simulink model "OR_10s_70l"  (R2023b)
settings: Solver=VariableStepAuto  StartTime=0.0  StopTime=10.0  RelTol=1e-3
undefined symbols (not defined in the file or in its folder): null
libraries: ABB_UPPAAL_Library x168
(part 1 of 3)
settings Model: Creator=francescopellei  LastModifiedBy=francescopellei

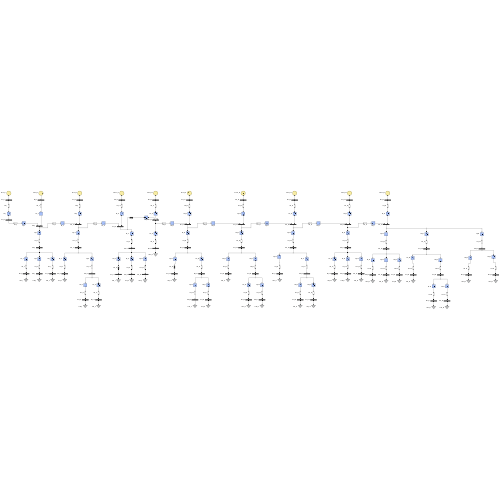
[thumbnail: Simulink's stored preview of the top-level diagram]
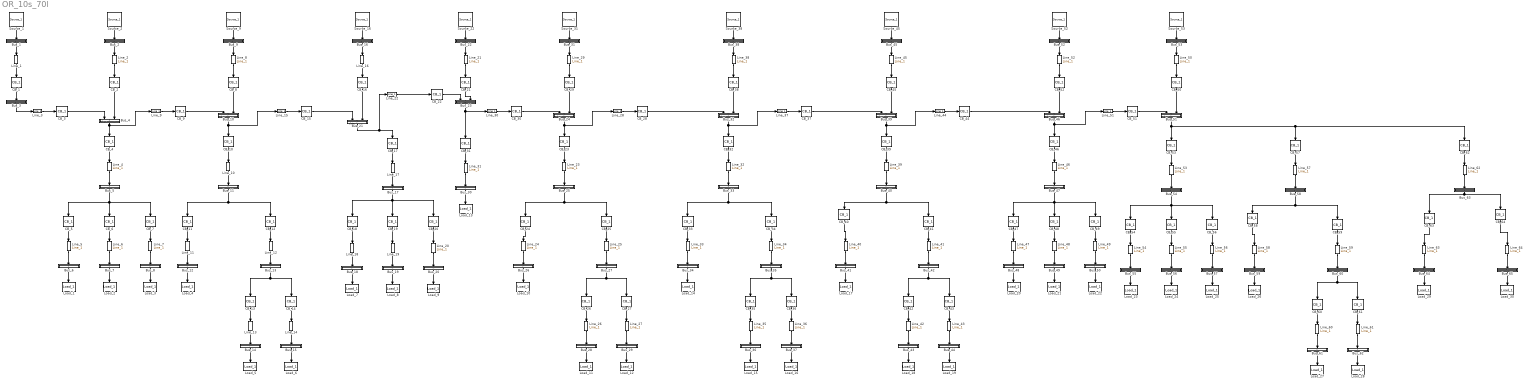
== system OR_10s_70l ==
  Bus_1 : MATLAB Function  TreatAsAtomicUnit=on  mask{MyInitialization=0, Bus_ID=1, Fault_flag=1}
      mask prompts: Bus_ID "Bus ID"; Fault_flag "Fault flag"
      settings: CopyFcn=|
      | Component_Name = get_param(gcb, 'Name');
      | set_param(gcb, 'Bus_ID', num2str(strtrim(extractAfter(Component_Name, '_'))));
      | 
      | blocks = find_system(gcs, 'SearchDepth', 1, 'Type', 'Block');
      | 
      | for k = 1:length(blocks)
      |     if contains(extractAfter(blocks{k,1}, '/'), 'Source')
      |         set_param(blocks{k}, 'BackgroundColor', '[0.929000, 0.490000, 0.439000]');
      |     end
      | end
      settings: NameChangeFcn=|
      | Component_Name = get_param(gcb, 'Name');
      | old_ID = get_param(gcb, 'Bus_ID');
      | 
      | pattern = '_\d+';
      | match = regexp(Component_Name, pattern, 'match');
      | 
      | if ~isempty(match)
      |     if ~isequal(old_ID, num2str(strtrim(extractAfter(Component_Name, '_'))))
      |         set_param(gcb, 'Bus_ID', num2str(strtrim(extractAfter(Component_Name, '_'))));
      |     end
      | else
      |     newName = [Component_Name '_' old_ID];
      |     set_param(gcb, 'Name', newName);
      | end
      | 
      | if ~isequal(old_ID, get_param(gcb, 'Bus_ID'))
      | 
      |     data = get_param(gcb, 'PortConnectivity');
      |     for i = 1:numel(data)
      |         sourceHandle = data(i,1).SrcBlock;
      |         if ~isempty(sourceHandle) && sourceHandle ~= -1
      |             sourceParams = get_param(sourceHandle, 'DialogParameters');
      |             fn = fieldnames(sourceParams);
      |             if contains(fn{2}, 'Source')
      |                 Bus_ID = get_param(gcb, 'Bus_ID');
      |                 set_param(sourceHandle, 'Source_ID', Bus_ID);
      |             end
      |         end
      |     end
      | 
      |     blocks = find_system(gcs, 'SearchDepth', 1, 'Type', 'Block');
      | 
      |     for k = 1:length(blocks)
      |         if contains(extractAfter(blocks{k,1}, '/'), 'Source')
      |             set_param(blocks{k}, 'BackgroundColor', '[0.929000, 0.490000, 0.439000]');
      |         end
      |     end
      | 
      | end
      settings: PreDeleteFcn=|
      | blocks = find_system(gcs, 'SearchDepth', 1, 'Type', 'Block');
      | 
      | for k = 1:length(blocks)
      |     if contains(extractAfter(blocks{k,1}, '/'), 'Source')
      |         set_param(blocks{k}, 'BackgroundColor', '[0.929000, 0.490000, 0.439000]');
      |     end
      | end
  Bus_10 : MATLAB Function  TreatAsAtomicUnit=on  mask{MyInitialization=0, Bus_ID=10, Fault_flag=1}
      mask prompts: Bus_ID "Bus ID"; Fault_flag "Fault flag"
      settings: CopyFcn=|
      | Component_Name = get_param(gcb, 'Name');
      | set_param(gcb, 'Bus_ID', num2str(strtrim(extractAfter(Component_Name, '_'))));
      | 
      | blocks = find_system(gcs, 'SearchDepth', 1, 'Type', 'Block');
      | 
      | for k = 1:length(blocks)
      |     if contains(extractAfter(blocks{k,1}, '/'), 'Source')
      |         set_param(blocks{k}, 'BackgroundColor', '[0.929000, 0.490000, 0.439000]');
      |     end
      | end
      settings: NameChangeFcn=|
      | Component_Name = get_param(gcb, 'Name');
      | old_ID = get_param(gcb, 'Bus_ID');
      | 
      | pattern = '_\d+';
      | match = regexp(Component_Name, pattern, 'match');
      | 
      | if ~isempty(match)
      |     if ~isequal(old_ID, num2str(strtrim(extractAfter(Component_Name, '_'))))
      |         set_param(gcb, 'Bus_ID', num2str(strtrim(extractAfter(Component_Name, '_'))));
      |     end
      | else
      |     newName = [Component_Name '_' old_ID];
      |     set_param(gcb, 'Name', newName);
      | end
      | 
      | if ~isequal(old_ID, get_param(gcb, 'Bus_ID'))
      | 
      |     data = get_param(gcb, 'PortConnectivity');
      |     for i = 1:numel(data)
      |         sourceHandle = data(i,1).SrcBlock;
      |         if ~isempty(sourceHandle) && sourceHandle ~= -1
      |             sourceParams = get_param(sourceHandle, 'DialogParameters');
      |             fn = fieldnames(sourceParams);
      |             if contains(fn{2}, 'Source')
      |                 Bus_ID = get_param(gcb, 'Bus_ID');
      |                 set_param(sourceHandle, 'Source_ID', Bus_ID);
      |             end
      |         end
      |     end
      | 
      |     blocks = find_system(gcs, 'SearchDepth', 1, 'Type', 'Block');
      | 
      |     for k = 1:length(blocks)
      |         if contains(extractAfter(blocks{k,1}, '/'), 'Source')
      |             set_param(blocks{k}, 'BackgroundColor', '[0.929000, 0.490000, 0.439000]');
      |         end
      |     end
      | 
      | end
      settings: PreDeleteFcn=|
      | blocks = find_system(gcs, 'SearchDepth', 1, 'Type', 'Block');
      | 
      | for k = 1:length(blocks)
      |     if contains(extractAfter(blocks{k,1}, '/'), 'Source')
      |         set_param(blocks{k}, 'BackgroundColor', '[0.929000, 0.490000, 0.439000]');
      |     end
      | end
  Bus_11 : MATLAB Function  TreatAsAtomicUnit=on  mask{MyInitialization=0, Bus_ID=11, Fault_flag=0}
      mask prompts: Bus_ID "Bus ID"; Fault_flag "Fault flag"
      settings: CopyFcn=|
      | Component_Name = get_param(gcb, 'Name');
      | set_param(gcb, 'Bus_ID', num2str(strtrim(extractAfter(Component_Name, '_'))));
      | 
      | blocks = find_system(gcs, 'SearchDepth', 1, 'Type', 'Block');
      | 
      | for k = 1:length(blocks)
      |     if contains(extractAfter(blocks{k,1}, '/'), 'Source')
      |         set_param(blocks{k}, 'BackgroundColor', '[0.929000, 0.490000, 0.439000]');
      |     end
      | end
      settings: NameChangeFcn=|
      | Component_Name = get_param(gcb, 'Name');
      | old_ID = get_param(gcb, 'Bus_ID');
      | 
      | pattern = '_\d+';
      | match = regexp(Component_Name, pattern, 'match');
      | 
      | if ~isempty(match)
      |     if ~isequal(old_ID, num2str(strtrim(extractAfter(Component_Name, '_'))))
      |         set_param(gcb, 'Bus_ID', num2str(strtrim(extractAfter(Component_Name, '_'))));
      |     end
      | else
      |     newName = [Component_Name '_' old_ID];
      |     set_param(gcb, 'Name', newName);
      | end
      | 
      | if ~isequal(old_ID, get_param(gcb, 'Bus_ID'))
      | 
      |     data = get_param(gcb, 'PortConnectivity');
      |     for i = 1:numel(data)
      |         sourceHandle = data(i,1).SrcBlock;
      |         if ~isempty(sourceHandle) && sourceHandle ~= -1
      |             sourceParams = get_param(sourceHandle, 'DialogParameters');
      |             fn = fieldnames(sourceParams);
      |             if contains(fn{2}, 'Source')
      |                 Bus_ID = get_param(gcb, 'Bus_ID');
      |                 set_param(sourceHandle, 'Source_ID', Bus_ID);
      |             end
      |         end
      |     end
      | 
      |     blocks = find_system(gcs, 'SearchDepth', 1, 'Type', 'Block');
      | 
      |     for k = 1:length(blocks)
      |         if contains(extractAfter(blocks{k,1}, '/'), 'Source')
      |             set_param(blocks{k}, 'BackgroundColor', '[0.929000, 0.490000, 0.439000]');
      |         end
      |     end
      | 
      | end
      settings: PreDeleteFcn=|
      | blocks = find_system(gcs, 'SearchDepth', 1, 'Type', 'Block');
      | 
      | for k = 1:length(blocks)
      |     if contains(extractAfter(blocks{k,1}, '/'), 'Source')
      |         set_param(blocks{k}, 'BackgroundColor', '[0.929000, 0.490000, 0.439000]');
      |     end
      | end
  Bus_12 : MATLAB Function  TreatAsAtomicUnit=on  mask{MyInitialization=0, Bus_ID=12, Fault_flag=1}
      mask prompts: Bus_ID "Bus ID"; Fault_flag "Fault flag"
      settings: CopyFcn=|
      | Component_Name = get_param(gcb, 'Name');
      | set_param(gcb, 'Bus_ID', num2str(strtrim(extractAfter(Component_Name, '_'))));
      | 
      | blocks = find_system(gcs, 'SearchDepth', 1, 'Type', 'Block');
      | 
      | for k = 1:length(blocks)
      |     if contains(extractAfter(blocks{k,1}, '/'), 'Source')
      |         set_param(blocks{k}, 'BackgroundColor', '[0.929000, 0.490000, 0.439000]');
      |     end
      | end
      settings: NameChangeFcn=|
      | Component_Name = get_param(gcb, 'Name');
      | old_ID = get_param(gcb, 'Bus_ID');
      | 
      | pattern = '_\d+';
      | match = regexp(Component_Name, pattern, 'match');
      | 
      | if ~isempty(match)
      |     if ~isequal(old_ID, num2str(strtrim(extractAfter(Component_Name, '_'))))
      |         set_param(gcb, 'Bus_ID', num2str(strtrim(extractAfter(Component_Name, '_'))));
      |     end
      | else
      |     newName = [Component_Name '_' old_ID];
      |     set_param(gcb, 'Name', newName);
      | end
      | 
      | if ~isequal(old_ID, get_param(gcb, 'Bus_ID'))
      | 
      |     data = get_param(gcb, 'PortConnectivity');
      |     for i = 1:numel(data)
      |         sourceHandle = data(i,1).SrcBlock;
      |         if ~isempty(sourceHandle) && sourceHandle ~= -1
      |             sourceParams = get_param(sourceHandle, 'DialogParameters');
      |             fn = fieldnames(sourceParams);
      |             if contains(fn{2}, 'Source')
      |                 Bus_ID = get_param(gcb, 'Bus_ID');
      |                 set_param(sourceHandle, 'Source_ID', Bus_ID);
      |             end
      |         end
      |     end
      | 
      |     blocks = find_system(gcs, 'SearchDepth', 1, 'Type', 'Block');
      | 
      |     for k = 1:length(blocks)
      |         if contains(extractAfter(blocks{k,1}, '/'), 'Source')
      |             set_param(blocks{k}, 'BackgroundColor', '[0.929000, 0.490000, 0.439000]');
      |         end
      |     end
      | 
      | end
      settings: PreDeleteFcn=|
      | blocks = find_system(gcs, 'SearchDepth', 1, 'Type', 'Block');
      | 
      | for k = 1:length(blocks)
      |     if contains(extractAfter(blocks{k,1}, '/'), 'Source')
      |         set_param(blocks{k}, 'BackgroundColor', '[0.929000, 0.490000, 0.439000]');
      |     end
      | end
  Bus_13 : MATLAB Function  TreatAsAtomicUnit=on  mask{MyInitialization=0, Bus_ID=13, Fault_flag=1}
      mask prompts: Bus_ID "Bus ID"; Fault_flag "Fault flag"
      settings: CopyFcn=|
      | Component_Name = get_param(gcb, 'Name');
      | set_param(gcb, 'Bus_ID', num2str(strtrim(extractAfter(Component_Name, '_'))));
      | 
      | blocks = find_system(gcs, 'SearchDepth', 1, 'Type', 'Block');
      | 
      | for k = 1:length(blocks)
      |     if contains(extractAfter(blocks{k,1}, '/'), 'Source')
      |         set_param(blocks{k}, 'BackgroundColor', '[0.929000, 0.490000, 0.439000]');
      |     end
      | end
      settings: NameChangeFcn=|
      | Component_Name = get_param(gcb, 'Name');
      | old_ID = get_param(gcb, 'Bus_ID');
      | 
      | pattern = '_\d+';
      | match = regexp(Component_Name, pattern, 'match');
      | 
      | if ~isempty(match)
      |     if ~isequal(old_ID, num2str(strtrim(extractAfter(Component_Name, '_'))))
      |         set_param(gcb, 'Bus_ID', num2str(strtrim(extractAfter(Component_Name, '_'))));
      |     end
      | else
      |     newName = [Component_Name '_' old_ID];
      |     set_param(gcb, 'Name', newName);
      | end
      | 
      | if ~isequal(old_ID, get_param(gcb, 'Bus_ID'))
      | 
      |     data = get_param(gcb, 'PortConnectivity');
      |     for i = 1:numel(data)
      |         sourceHandle = data(i,1).SrcBlock;
      |         if ~isempty(sourceHandle) && sourceHandle ~= -1
      |             sourceParams = get_param(sourceHandle, 'DialogParameters');
      |             fn = fieldnames(sourceParams);
      |             if contains(fn{2}, 'Source')
      |                 Bus_ID = get_param(gcb, 'Bus_ID');
      |                 set_param(sourceHandle, 'Source_ID', Bus_ID);
      |             end
      |         end
      |     end
      | 
      |     blocks = find_system(gcs, 'SearchDepth', 1, 'Type', 'Block');
      | 
      |     for k = 1:length(blocks)
      |         if contains(extractAfter(blocks{k,1}, '/'), 'Source')
      |             set_param(blocks{k}, 'BackgroundColor', '[0.929000, 0.490000, 0.439000]');
      |         end
      |     end
      | 
      | end
      settings: PreDeleteFcn=|
      | blocks = find_system(gcs, 'SearchDepth', 1, 'Type', 'Block');
      | 
      | for k = 1:length(blocks)
      |     if contains(extractAfter(blocks{k,1}, '/'), 'Source')
      |         set_param(blocks{k}, 'BackgroundColor', '[0.929000, 0.490000, 0.439000]');
      |     end
      | end
  Bus_14 : MATLAB Function  TreatAsAtomicUnit=on  mask{MyInitialization=0, Bus_ID=14, Fault_flag=1}
      mask prompts: Bus_ID "Bus ID"; Fault_flag "Fault flag"
      settings: CopyFcn=|
      | Component_Name = get_param(gcb, 'Name');
      | set_param(gcb, 'Bus_ID', num2str(strtrim(extractAfter(Component_Name, '_'))));
      | 
      | blocks = find_system(gcs, 'SearchDepth', 1, 'Type', 'Block');
      | 
      | for k = 1:length(blocks)
      |     if contains(extractAfter(blocks{k,1}, '/'), 'Source')
      |         set_param(blocks{k}, 'BackgroundColor', '[0.929000, 0.490000, 0.439000]');
      |     end
      | end
      settings: NameChangeFcn=|
      | Component_Name = get_param(gcb, 'Name');
      | old_ID = get_param(gcb, 'Bus_ID');
      | 
      | pattern = '_\d+';
      | match = regexp(Component_Name, pattern, 'match');
      | 
      | if ~isempty(match)
      |     if ~isequal(old_ID, num2str(strtrim(extractAfter(Component_Name, '_'))))
      |         set_param(gcb, 'Bus_ID', num2str(strtrim(extractAfter(Component_Name, '_'))));
      |     end
      | else
      |     newName = [Component_Name '_' old_ID];
      |     set_param(gcb, 'Name', newName);
      | end
      | 
      | if ~isequal(old_ID, get_param(gcb, 'Bus_ID'))
      | 
      |     data = get_param(gcb, 'PortConnectivity');
      |     for i = 1:numel(data)
      |         sourceHandle = data(i,1).SrcBlock;
      |         if ~isempty(sourceHandle) && sourceHandle ~= -1
      |             sourceParams = get_param(sourceHandle, 'DialogParameters');
      |             fn = fieldnames(sourceParams);
      |             if contains(fn{2}, 'Source')
      |                 Bus_ID = get_param(gcb, 'Bus_ID');
      |                 set_param(sourceHandle, 'Source_ID', Bus_ID);
      |             end
      |         end
      |     end
      | 
      |     blocks = find_system(gcs, 'SearchDepth', 1, 'Type', 'Block');
      | 
      |     for k = 1:length(blocks)
      |         if contains(extractAfter(blocks{k,1}, '/'), 'Source')
      |             set_param(blocks{k}, 'BackgroundColor', '[0.929000, 0.490000, 0.439000]');
      |         end
      |     end
      | 
      | end
      settings: PreDeleteFcn=|
      | blocks = find_system(gcs, 'SearchDepth', 1, 'Type', 'Block');
      | 
      | for k = 1:length(blocks)
      |     if contains(extractAfter(blocks{k,1}, '/'), 'Source')
      |         set_param(blocks{k}, 'BackgroundColor', '[0.929000, 0.490000, 0.439000]');
      |     end
      | end
  Bus_15 : MATLAB Function  TreatAsAtomicUnit=on  mask{MyInitialization=0, Bus_ID=15, Fault_flag=1}
      mask prompts: Bus_ID "Bus ID"; Fault_flag "Fault flag"
      settings: CopyFcn=|
      | Component_Name = get_param(gcb, 'Name');
      | set_param(gcb, 'Bus_ID', num2str(strtrim(extractAfter(Component_Name, '_'))));
      | 
      | blocks = find_system(gcs, 'SearchDepth', 1, 'Type', 'Block');
      | 
      | for k = 1:length(blocks)
      |     if contains(extractAfter(blocks{k,1}, '/'), 'Source')
      |         set_param(blocks{k}, 'BackgroundColor', '[0.929000, 0.490000, 0.439000]');
      |     end
      | end
      settings: NameChangeFcn=|
      | Component_Name = get_param(gcb, 'Name');
      | old_ID = get_param(gcb, 'Bus_ID');
      | 
      | pattern = '_\d+';
      | match = regexp(Component_Name, pattern, 'match');
      | 
      | if ~isempty(match)
      |     if ~isequal(old_ID, num2str(strtrim(extractAfter(Component_Name, '_'))))
      |         set_param(gcb, 'Bus_ID', num2str(strtrim(extractAfter(Component_Name, '_'))));
      |     end
      | else
      |     newName = [Component_Name '_' old_ID];
      |     set_param(gcb, 'Name', newName);
      | end
      | 
      | if ~isequal(old_ID, get_param(gcb, 'Bus_ID'))
      | 
      |     data = get_param(gcb, 'PortConnectivity');
      |     for i = 1:numel(data)
      |         sourceHandle = data(i,1).SrcBlock;
      |         if ~isempty(sourceHandle) && sourceHandle ~= -1
      |             sourceParams = get_param(sourceHandle, 'DialogParameters');
      |             fn = fieldnames(sourceParams);
      |             if contains(fn{2}, 'Source')
      |                 Bus_ID = get_param(gcb, 'Bus_ID');
      |                 set_param(sourceHandle, 'Source_ID', Bus_ID);
      |             end
      |         end
      |     end
      | 
      |     blocks = find_system(gcs, 'SearchDepth', 1, 'Type', 'Block');
      | 
      |     for k = 1:length(blocks)
      |         if contains(extractAfter(blocks{k,1}, '/'), 'Source')
      |             set_param(blocks{k}, 'BackgroundColor', '[0.929000, 0.490000, 0.439000]');
      |         end
      |     end
      | 
      | end
      settings: PreDeleteFcn=|
      | blocks = find_system(gcs, 'SearchDepth', 1, 'Type', 'Block');
      | 
      | for k = 1:length(blocks)
      |     if contains(extractAfter(blocks{k,1}, '/'), 'Source')
      |         set_param(blocks{k}, 'BackgroundColor', '[0.929000, 0.490000, 0.439000]');
      |     end
      | end
  Bus_16 : MATLAB Function  TreatAsAtomicUnit=on  mask{MyInitialization=0, Bus_ID=16, Fault_flag=1}
      mask prompts: Bus_ID "Bus ID"; Fault_flag "Fault flag"
      settings: CopyFcn=|
      | Component_Name = get_param(gcb, 'Name');
      | set_param(gcb, 'Bus_ID', num2str(strtrim(extractAfter(Component_Name, '_'))));
      | 
      | blocks = find_system(gcs, 'SearchDepth', 1, 'Type', 'Block');
      | 
      | for k = 1:length(blocks)
      |     if contains(extractAfter(blocks{k,1}, '/'), 'Source')
      |         set_param(blocks{k}, 'BackgroundColor', '[0.929000, 0.490000, 0.439000]');
      |     end
      | end
      settings: NameChangeFcn=|
      | Component_Name = get_param(gcb, 'Name');
      | old_ID = get_param(gcb, 'Bus_ID');
      | 
      | pattern = '_\d+';
      | match = regexp(Component_Name, pattern, 'match');
      | 
      | if ~isempty(match)
      |     if ~isequal(old_ID, num2str(strtrim(extractAfter(Component_Name, '_'))))
      |         set_param(gcb, 'Bus_ID', num2str(strtrim(extractAfter(Component_Name, '_'))));
      |     end
      | else
      |     newName = [Component_Name '_' old_ID];
      |     set_param(gcb, 'Name', newName);
      | end
      | 
      | if ~isequal(old_ID, get_param(gcb, 'Bus_ID'))
      | 
      |     data = get_param(gcb, 'PortConnectivity');
      |     for i = 1:numel(data)
      |         sourceHandle = data(i,1).SrcBlock;
      |         if ~isempty(sourceHandle) && sourceHandle ~= -1
      |             sourceParams = get_param(sourceHandle, 'DialogParameters');
      |             fn = fieldnames(sourceParams);
      |             if contains(fn{2}, 'Source')
      |                 Bus_ID = get_param(gcb, 'Bus_ID');
      |                 set_param(sourceHandle, 'Source_ID', Bus_ID);
      |             end
      |         end
      |     end
      | 
      |     blocks = find_system(gcs, 'SearchDepth', 1, 'Type', 'Block');
      | 
      |     for k = 1:length(blocks)
      |         if contains(extractAfter(blocks{k,1}, '/'), 'Source')
      |             set_param(blocks{k}, 'BackgroundColor', '[0.929000, 0.490000, 0.439000]');
      |         end
      |     end
      | 
      | end
      settings: PreDeleteFcn=|
      | blocks = find_system(gcs, 'SearchDepth', 1, 'Type', 'Block');
      | 
      | for k = 1:length(blocks)
      |     if contains(extractAfter(blocks{k,1}, '/'), 'Source')
      |         set_param(blocks{k}, 'BackgroundColor', '[0.929000, 0.490000, 0.439000]');
      |     end
      | end
  Bus_17 : MATLAB Function  TreatAsAtomicUnit=on  mask{MyInitialization=0, Bus_ID=17, Fault_flag=1}
      mask prompts: Bus_ID "Bus ID"; Fault_flag "Fault flag"
      settings: CopyFcn=|
      | Component_Name = get_param(gcb, 'Name');
      | set_param(gcb, 'Bus_ID', num2str(strtrim(extractAfter(Component_Name, '_'))));
      | 
      | blocks = find_system(gcs, 'SearchDepth', 1, 'Type', 'Block');
      | 
      | for k = 1:length(blocks)
      |     if contains(extractAfter(blocks{k,1}, '/'), 'Source')
      |         set_param(blocks{k}, 'BackgroundColor', '[0.929000, 0.490000, 0.439000]');
      |     end
      | end
      settings: NameChangeFcn=|
      | Component_Name = get_param(gcb, 'Name');
      | old_ID = get_param(gcb, 'Bus_ID');
      | 
      | pattern = '_\d+';
      | match = regexp(Component_Name, pattern, 'match');
      | 
      | if ~isempty(match)
      |     if ~isequal(old_ID, num2str(strtrim(extractAfter(Component_Name, '_'))))
      |         set_param(gcb, 'Bus_ID', num2str(strtrim(extractAfter(Component_Name, '_'))));
      |     end
      | else
      |     newName = [Component_Name '_' old_ID];
      |     set_param(gcb, 'Name', newName);
      | end
      | 
      | if ~isequal(old_ID, get_param(gcb, 'Bus_ID'))
      | 
      |     data = get_param(gcb, 'PortConnectivity');
      |     for i = 1:numel(data)
      |         sourceHandle = data(i,1).SrcBlock;
      |         if ~isempty(sourceHandle) && sourceHandle ~= -1
      |             sourceParams = get_param(sourceHandle, 'DialogParameters');
      |             fn = fieldnames(sourceParams);
      |             if contains(fn{2}, 'Source')
      |                 Bus_ID = get_param(gcb, 'Bus_ID');
      |                 set_param(sourceHandle, 'Source_ID', Bus_ID);
      |             end
      |         end
      |     end
      | 
      |     blocks = find_system(gcs, 'SearchDepth', 1, 'Type', 'Block');
      | 
      |     for k = 1:length(blocks)
      |         if contains(extractAfter(blocks{k,1}, '/'), 'Source')
      |             set_param(blocks{k}, 'BackgroundColor', '[0.929000, 0.490000, 0.439000]');
      |         end
      |     end
      | 
      | end
      settings: PreDeleteFcn=|
      | blocks = find_system(gcs, 'SearchDepth', 1, 'Type', 'Block');
      | 
      | for k = 1:length(blocks)
      |     if contains(extractAfter(blocks{k,1}, '/'), 'Source')
      |         set_param(blocks{k}, 'BackgroundColor', '[0.929000, 0.490000, 0.439000]');
      |     end
      | end
  Bus_18 : MATLAB Function  TreatAsAtomicUnit=on  mask{MyInitialization=0, Bus_ID=18, Fault_flag=1}
      mask prompts: Bus_ID "Bus ID"; Fault_flag "Fault flag"
      settings: CopyFcn=|
      | Component_Name = get_param(gcb, 'Name');
      | set_param(gcb, 'Bus_ID', num2str(strtrim(extractAfter(Component_Name, '_'))));
      | 
      | blocks = find_system(gcs, 'SearchDepth', 1, 'Type', 'Block');
      | 
      | for k = 1:length(blocks)
      |     if contains(extractAfter(blocks{k,1}, '/'), 'Source')
      |         set_param(blocks{k}, 'BackgroundColor', '[0.929000, 0.490000, 0.439000]');
      |     end
      | end
      settings: NameChangeFcn=|
      | Component_Name = get_param(gcb, 'Name');
      | old_ID = get_param(gcb, 'Bus_ID');
      | 
      | pattern = '_\d+';
      | match = regexp(Component_Name, pattern, 'match');
      | 
      | if ~isempty(match)
      |     if ~isequal(old_ID, num2str(strtrim(extractAfter(Component_Name, '_'))))
      |         set_param(gcb, 'Bus_ID', num2str(strtrim(extractAfter(Component_Name, '_'))));
      |     end
      | else
      |     newName = [Component_Name '_' old_ID];
      |     set_param(gcb, 'Name', newName);
      | end
      | 
      | if ~isequal(old_ID, get_param(gcb, 'Bus_ID'))
      | 
      |     data = get_param(gcb, 'PortConnectivity');
      |     for i = 1:numel(data)
      |         sourceHandle = data(i,1).SrcBlock;
      |         if ~isempty(sourceHandle) && sourceHandle ~= -1
      |             sourceParams = get_param(sourceHandle, 'DialogParameters');
      |             fn = fieldnames(sourceParams);
      |             if contains(fn{2}, 'Source')
      |                 Bus_ID = get_param(gcb, 'Bus_ID');
      |                 set_param(sourceHandle, 'Source_ID', Bus_ID);
      |             end
      |         end
      |     end
      | 
      |     blocks = find_system(gcs, 'SearchDepth', 1, 'Type', 'Block');
      | 
      |     for k = 1:length(blocks)
      |         if contains(extractAfter(blocks{k,1}, '/'), 'Source')
      |             set_param(blocks{k}, 'BackgroundColor', '[0.929000, 0.490000, 0.439000]');
      |         end
      |     end
      | 
      | end
      settings: PreDeleteFcn=|
      | blocks = find_system(gcs, 'SearchDepth', 1, 'Type', 'Block');
      | 
      | for k = 1:length(blocks)
      |     if contains(extractAfter(blocks{k,1}, '/'), 'Source')
      |         set_param(blocks{k}, 'BackgroundColor', '[0.929000, 0.490000, 0.439000]');
      |     end
      | end
  Bus_19 : MATLAB Function  TreatAsAtomicUnit=on  mask{MyInitialization=0, Bus_ID=19, Fault_flag=0}
      mask prompts: Bus_ID "Bus ID"; Fault_flag "Fault flag"
      settings: CopyFcn=|
      | Component_Name = get_param(gcb, 'Name');
      | set_param(gcb, 'Bus_ID', num2str(strtrim(extractAfter(Component_Name, '_'))));
      | 
      | blocks = find_system(gcs, 'SearchDepth', 1, 'Type', 'Block');
      | 
      | for k = 1:length(blocks)
      |     if contains(extractAfter(blocks{k,1}, '/'), 'Source')
      |         set_param(blocks{k}, 'BackgroundColor', '[0.929000, 0.490000, 0.439000]');
      |     end
      | end
      settings: NameChangeFcn=|
      | Component_Name = get_param(gcb, 'Name');
      | old_ID = get_param(gcb, 'Bus_ID');
      | 
      | pattern = '_\d+';
      | match = regexp(Component_Name, pattern, 'match');
      | 
      | if ~isempty(match)
      |     if ~isequal(old_ID, num2str(strtrim(extractAfter(Component_Name, '_'))))
      |         set_param(gcb, 'Bus_ID', num2str(strtrim(extractAfter(Component_Name, '_'))));
      |     end
      | else
      |     newName = [Component_Name '_' old_ID];
      |     set_param(gcb, 'Name', newName);
      | end
      | 
      | if ~isequal(old_ID, get_param(gcb, 'Bus_ID'))
      | 
      |     data = get_param(gcb, 'PortConnectivity');
      |     for i = 1:numel(data)
      |         sourceHandle = data(i,1).SrcBlock;
      |         if ~isempty(sourceHandle) && sourceHandle ~= -1
      |             sourceParams = get_param(sourceHandle, 'DialogParameters');
      |             fn = fieldnames(sourceParams);
      |             if contains(fn{2}, 'Source')
      |                 Bus_ID = get_param(gcb, 'Bus_ID');
      |                 set_param(sourceHandle, 'Source_ID', Bus_ID);
      |             end
      |         end
      |     end
      | 
      |     blocks = find_system(gcs, 'SearchDepth', 1, 'Type', 'Block');
      | 
      |     for k = 1:length(blocks)
      |         if contains(extractAfter(blocks{k,1}, '/'), 'Source')
      |             set_param(blocks{k}, 'BackgroundColor', '[0.929000, 0.490000, 0.439000]');
      |         end
      |     end
      | 
      | end
      settings: PreDeleteFcn=|
      | blocks = find_system(gcs, 'SearchDepth', 1, 'Type', 'Block');
      | 
      | for k = 1:length(blocks)
      |     if contains(extractAfter(blocks{k,1}, '/'), 'Source')
      |         set_param(blocks{k}, 'BackgroundColor', '[0.929000, 0.490000, 0.439000]');
      |     end
      | end
  Bus_2 : MATLAB Function  TreatAsAtomicUnit=on  mask{MyInitialization=0, Bus_ID=2, Fault_flag=1}
      mask prompts: Bus_ID "Bus ID"; Fault_flag "Fault flag"
      settings: CopyFcn=|
      | Component_Name = get_param(gcb, 'Name');
      | set_param(gcb, 'Bus_ID', num2str(strtrim(extractAfter(Component_Name, '_'))));
      | 
      | blocks = find_system(gcs, 'SearchDepth', 1, 'Type', 'Block');
      | 
      | for k = 1:length(blocks)
      |     if contains(extractAfter(blocks{k,1}, '/'), 'Source')
      |         set_param(blocks{k}, 'BackgroundColor', '[0.929000, 0.490000, 0.439000]');
      |     end
      | end
      settings: NameChangeFcn=|
      | Component_Name = get_param(gcb, 'Name');
      | old_ID = get_param(gcb, 'Bus_ID');
      | 
      | pattern = '_\d+';
      | match = regexp(Component_Name, pattern, 'match');
      | 
      | if ~isempty(match)
      |     if ~isequal(old_ID, num2str(strtrim(extractAfter(Component_Name, '_'))))
      |         set_param(gcb, 'Bus_ID', num2str(strtrim(extractAfter(Component_Name, '_'))));
      |     end
      | else
      |     newName = [Component_Name '_' old_ID];
      |     set_param(gcb, 'Name', newName);
      | end
      | 
      | if ~isequal(old_ID, get_param(gcb, 'Bus_ID'))
      | 
      |     data = get_param(gcb, 'PortConnectivity');
      |     for i = 1:numel(data)
      |         sourceHandle = data(i,1).SrcBlock;
      |         if ~isempty(sourceHandle) && sourceHandle ~= -1
      |             sourceParams = get_param(sourceHandle, 'DialogParameters');
      |             fn = fieldnames(sourceParams);
      |             if contains(fn{2}, 'Source')
      |                 Bus_ID = get_param(gcb, 'Bus_ID');
      |                 set_param(sourceHandle, 'Source_ID', Bus_ID);
      |             end
      |         end
      |     end
      | 
      |     blocks = find_system(gcs, 'SearchDepth', 1, 'Type', 'Block');
      | 
      |     for k = 1:length(blocks)
      |         if contains(extractAfter(blocks{k,1}, '/'), 'Source')
      |             set_param(blocks{k}, 'BackgroundColor', '[0.929000, 0.490000, 0.439000]');
      |         end
      |     end
      | 
      | end
      settings: PreDeleteFcn=|
      | blocks = find_system(gcs, 'SearchDepth', 1, 'Type', 'Block');
      | 
      | for k = 1:length(blocks)
      |     if contains(extractAfter(blocks{k,1}, '/'), 'Source')
      |         set_param(blocks{k}, 'BackgroundColor', '[0.929000, 0.490000, 0.439000]');
      |     end
      | end
  Bus_20 : MATLAB Function  TreatAsAtomicUnit=on  mask{MyInitialization=0, Bus_ID=20, Fault_flag=1}
      mask prompts: Bus_ID "Bus ID"; Fault_flag "Fault flag"
      settings: CopyFcn=|
      | Component_Name = get_param(gcb, 'Name');
      | set_param(gcb, 'Bus_ID', num2str(strtrim(extractAfter(Component_Name, '_'))));
      | 
      | blocks = find_system(gcs, 'SearchDepth', 1, 'Type', 'Block');
      | 
      | for k = 1:length(blocks)
      |     if contains(extractAfter(blocks{k,1}, '/'), 'Source')
      |         set_param(blocks{k}, 'BackgroundColor', '[0.929000, 0.490000, 0.439000]');
      |     end
      | end
      settings: NameChangeFcn=|
      | Component_Name = get_param(gcb, 'Name');
      | old_ID = get_param(gcb, 'Bus_ID');
      | 
      | pattern = '_\d+';
      | match = regexp(Component_Name, pattern, 'match');
      | 
      | if ~isempty(match)
      |     if ~isequal(old_ID, num2str(strtrim(extractAfter(Component_Name, '_'))))
      |         set_param(gcb, 'Bus_ID', num2str(strtrim(extractAfter(Component_Name, '_'))));
      |     end
      | else
      |     newName = [Component_Name '_' old_ID];
      |     set_param(gcb, 'Name', newName);
      | end
      | 
      | if ~isequal(old_ID, get_param(gcb, 'Bus_ID'))
      | 
      |     data = get_param(gcb, 'PortConnectivity');
      |     for i = 1:numel(data)
      |         sourceHandle = data(i,1).SrcBlock;
      |         if ~isempty(sourceHandle) && sourceHandle ~= -1
      |             sourceParams = get_param(sourceHandle, 'DialogParameters');
      |             fn = fieldnames(sourceParams);
      |             if contains(fn{2}, 'Source')
      |                 Bus_ID = get_param(gcb, 'Bus_ID');
      |                 set_param(sourceHandle, 'Source_ID', Bus_ID);
      |             end
      |         end
      |     end
      | 
      |     blocks = find_system(gcs, 'SearchDepth', 1, 'Type', 'Block');
      | 
      |     for k = 1:length(blocks)
      |         if contains(extractAfter(blocks{k,1}, '/'), 'Source')
      |             set_param(blocks{k}, 'BackgroundColor', '[0.929000, 0.490000, 0.439000]');
      |         end
      |     end
      | 
      | end
      settings: PreDeleteFcn=|
      | blocks = find_system(gcs, 'SearchDepth', 1, 'Type', 'Block');
      | 
      | for k = 1:length(blocks)
      |     if contains(extractAfter(blocks{k,1}, '/'), 'Source')
      |         set_param(blocks{k}, 'BackgroundColor', '[0.929000, 0.490000, 0.439000]');
      |     end
      | end
  Bus_21 : MATLAB Function  TreatAsAtomicUnit=on  mask{MyInitialization=0, Bus_ID=21, Fault_flag=1}
      mask prompts: Bus_ID "Bus ID"; Fault_flag "Fault flag"
      settings: CopyFcn=|
      | Component_Name = get_param(gcb, 'Name');
      | set_param(gcb, 'Bus_ID', num2str(strtrim(extractAfter(Component_Name, '_'))));
      | 
      | blocks = find_system(gcs, 'SearchDepth', 1, 'Type', 'Block');
      | 
      | for k = 1:length(blocks)
      |     if contains(extractAfter(blocks{k,1}, '/'), 'Source')
      |         set_param(blocks{k}, 'BackgroundColor', '[0.929000, 0.490000, 0.439000]');
      |     end
      | end
      settings: NameChangeFcn=|
      | Component_Name = get_param(gcb, 'Name');
      | old_ID = get_param(gcb, 'Bus_ID');
      | 
      | pattern = '_\d+';
      | match = regexp(Component_Name, pattern, 'match');
      | 
      | if ~isempty(match)
      |     if ~isequal(old_ID, num2str(strtrim(extractAfter(Component_Name, '_'))))
      |         set_param(gcb, 'Bus_ID', num2str(strtrim(extractAfter(Component_Name, '_'))));
      |     end
      | else
      |     newName = [Component_Name '_' old_ID];
      |     set_param(gcb, 'Name', newName);
      | end
      | 
      | if ~isequal(old_ID, get_param(gcb, 'Bus_ID'))
      | 
      |     data = get_param(gcb, 'PortConnectivity');
      |     for i = 1:numel(data)
      |         sourceHandle = data(i,1).SrcBlock;
      |         if ~isempty(sourceHandle) && sourceHandle ~= -1
      |             sourceParams = get_param(sourceHandle, 'DialogParameters');
      |             fn = fieldnames(sourceParams);
      |             if contains(fn{2}, 'Source')
      |                 Bus_ID = get_param(gcb, 'Bus_ID');
      |                 set_param(sourceHandle, 'Source_ID', Bus_ID);
      |             end
      |         end
      |     end
      | 
      |     blocks = find_system(gcs, 'SearchDepth', 1, 'Type', 'Block');
      | 
      |     for k = 1:length(blocks)
      |         if contains(extractAfter(blocks{k,1}, '/'), 'Source')
      |             set_param(blocks{k}, 'BackgroundColor', '[0.929000, 0.490000, 0.439000]');
      |         end
      |     end
      | 
      | end
      settings: PreDeleteFcn=|
      | blocks = find_system(gcs, 'SearchDepth', 1, 'Type', 'Block');
      | 
      | for k = 1:length(blocks)
      |     if contains(extractAfter(blocks{k,1}, '/'), 'Source')
      |         set_param(blocks{k}, 'BackgroundColor', '[0.929000, 0.490000, 0.439000]');
      |     end
      | end
  Bus_22 : MATLAB Function  TreatAsAtomicUnit=on  mask{MyInitialization=0, Bus_ID=22, Fault_flag=1}
      mask prompts: Bus_ID "Bus ID"; Fault_flag "Fault flag"
      settings: CopyFcn=|
      | Component_Name = get_param(gcb, 'Name');
      | set_param(gcb, 'Bus_ID', num2str(strtrim(extractAfter(Component_Name, '_'))));
      | 
      | blocks = find_system(gcs, 'SearchDepth', 1, 'Type', 'Block');
      | 
      | for k = 1:length(blocks)
      |     if contains(extractAfter(blocks{k,1}, '/'), 'Source')
      |         set_param(blocks{k}, 'BackgroundColor', '[0.929000, 0.490000, 0.439000]');
      |     end
      | end
      settings: NameChangeFcn=|
      | Component_Name = get_param(gcb, 'Name');
      | old_ID = get_param(gcb, 'Bus_ID');
      | 
      | pattern = '_\d+';
      | match = regexp(Component_Name, pattern, 'match');
      | 
      | if ~isempty(match)
      |     if ~isequal(old_ID, num2str(strtrim(extractAfter(Component_Name, '_'))))
      |         set_param(gcb, 'Bus_ID', num2str(strtrim(extractAfter(Component_Name, '_'))));
      |     end
      | else
      |     newName = [Component_Name '_' old_ID];
      |     set_param(gcb, 'Name', newName);
      | end
      | 
      | if ~isequal(old_ID, get_param(gcb, 'Bus_ID'))
      | 
      |     data = get_param(gcb, 'PortConnectivity');
      |     for i = 1:numel(data)
      |         sourceHandle = data(i,1).SrcBlock;
      |         if ~isempty(sourceHandle) && sourceHandle ~= -1
      |             sourceParams = get_param(sourceHandle, 'DialogParameters');
      |             fn = fieldnames(sourceParams);
      |             if contains(fn{2}, 'Source')
      |                 Bus_ID = get_param(gcb, 'Bus_ID');
      |                 set_param(sourceHandle, 'Source_ID', Bus_ID);
      |             end
      |         end
      |     end
      | 
      |     blocks = find_system(gcs, 'SearchDepth', 1, 'Type', 'Block');
      | 
      |     for k = 1:length(blocks)
      |         if contains(extractAfter(blocks{k,1}, '/'), 'Source')
      |             set_param(blocks{k}, 'BackgroundColor', '[0.929000, 0.490000, 0.439000]');
      |         end
      |     end
      | 
      | end
      settings: PreDeleteFcn=|
      | blocks = find_system(gcs, 'SearchDepth', 1, 'Type', 'Block');
      | 
      | for k = 1:length(blocks)
      |     if contains(extractAfter(blocks{k,1}, '/'), 'Source')
      |         set_param(blocks{k}, 'BackgroundColor', '[0.929000, 0.490000, 0.439000]');
      |     end
      | end
  Bus_23 : MATLAB Function  TreatAsAtomicUnit=on  mask{MyInitialization=0, Bus_ID=23, Fault_flag=1}
      mask prompts: Bus_ID "Bus ID"; Fault_flag "Fault flag"
      settings: CopyFcn=|
      | Component_Name = get_param(gcb, 'Name');
      | set_param(gcb, 'Bus_ID', num2str(strtrim(extractAfter(Component_Name, '_'))));
      | 
      | blocks = find_system(gcs, 'SearchDepth', 1, 'Type', 'Block');
      | 
      | for k = 1:length(blocks)
      |     if contains(extractAfter(blocks{k,1}, '/'), 'Source')
      |         set_param(blocks{k}, 'BackgroundColor', '[0.929000, 0.490000, 0.439000]');
      |     end
      | end
      settings: NameChangeFcn=|
      | Component_Name = get_param(gcb, 'Name');
      | old_ID = get_param(gcb, 'Bus_ID');
      | 
      | pattern = '_\d+';
      | match = regexp(Component_Name, pattern, 'match');
      | 
      | if ~isempty(match)
      |     if ~isequal(old_ID, num2str(strtrim(extractAfter(Component_Name, '_'))))
      |         set_param(gcb, 'Bus_ID', num2str(strtrim(extractAfter(Component_Name, '_'))));
      |     end
      | else
      |     newName = [Component_Name '_' old_ID];
      |     set_param(gcb, 'Name', newName);
      | end
      | 
      | if ~isequal(old_ID, get_param(gcb, 'Bus_ID'))
      | 
      |     data = get_param(gcb, 'PortConnectivity');
      |     for i = 1:numel(data)
      |         sourceHandle = data(i,1).SrcBlock;
      |         if ~isempty(sourceHandle) && sourceHandle ~= -1
      |             sourceParams = get_param(sourceHandle, 'DialogParameters');
      |             fn = fieldnames(sourceParams);
      |             if contains(fn{2}, 'Source')
      |                 Bus_ID = get_param(gcb, 'Bus_ID');
      |                 set_param(sourceHandle, 'Source_ID', Bus_ID);
      |             end
      |         end
      |     end
      | 
      |     blocks = find_system(gcs, 'SearchDepth', 1, 'Type', 'Block');
      | 
      |     for k = 1:length(blocks)
      |         if contains(extractAfter(blocks{k,1}, '/'), 'Source')
      |             set_param(blocks{k}, 'BackgroundColor', '[0.929000, 0.490000, 0.439000]');
      |         end
      |     end
      | 
      | end
      settings: PreDeleteFcn=|
      | blocks = find_system(gcs, 'SearchDepth', 1, 'Type', 'Block');
      | 
      | for k = 1:length(blocks)
      |     if contains(extractAfter(blocks{k,1}, '/'), 'Source')
      |         set_param(blocks{k}, 'BackgroundColor', '[0.929000, 0.490000, 0.439000]');
      |     end
      | end
  Bus_24 : MATLAB Function  TreatAsAtomicUnit=on  mask{MyInitialization=0, Bus_ID=24, Fault_flag=1}
      mask prompts: Bus_ID "Bus ID"; Fault_flag "Fault flag"
      settings: CopyFcn=|
      | Component_Name = get_param(gcb, 'Name');
      | set_param(gcb, 'Bus_ID', num2str(strtrim(extractAfter(Component_Name, '_'))));
      | 
      | blocks = find_system(gcs, 'SearchDepth', 1, 'Type', 'Block');
      | 
      | for k = 1:length(blocks)
      |     if contains(extractAfter(blocks{k,1}, '/'), 'Source')
      |         set_param(blocks{k}, 'BackgroundColor', '[0.929000, 0.490000, 0.439000]');
      |     end
      | end
      settings: NameChangeFcn=|
      | Component_Name = get_param(gcb, 'Name');
      | old_ID = get_param(gcb, 'Bus_ID');
      | 
      | pattern = '_\d+';
      | match = regexp(Component_Name, pattern, 'match');
      | 
      | if ~isempty(match)
      |     if ~isequal(old_ID, num2str(strtrim(extractAfter(Component_Name, '_'))))
      |         set_param(gcb, 'Bus_ID', num2str(strtrim(extractAfter(Component_Name, '_'))));
      |     end
      | else
      |     newName = [Component_Name '_' old_ID];
      |     set_param(gcb, 'Name', newName);
      | end
      | 
      | if ~isequal(old_ID, get_param(gcb, 'Bus_ID'))
      | 
      |     data = get_param(gcb, 'PortConnectivity');
      |     for i = 1:numel(data)
      |         sourceHandle = data(i,1).SrcBlock;
      |         if ~isempty(sourceHandle) && sourceHandle ~= -1
      |             sourceParams = get_param(sourceHandle, 'DialogParameters');
      |             fn = fieldnames(sourceParams);
      |             if contains(fn{2}, 'Source')
      |                 Bus_ID = get_param(gcb, 'Bus_ID');
      |                 set_param(sourceHandle, 'Source_ID', Bus_ID);
      |             end
      |         end
      |     end
      | 
      |     blocks = find_system(gcs, 'SearchDepth', 1, 'Type', 'Block');
      | 
      |     for k = 1:length(blocks)
      |         if contains(extractAfter(blocks{k,1}, '/'), 'Source')
      |             set_param(blocks{k}, 'BackgroundColor', '[0.929000, 0.490000, 0.439000]');
      |         end
      |     end
      | 
      | end
      settings: PreDeleteFcn=|
      | blocks = find_system(gcs, 'SearchDepth', 1, 'Type', 'Block');
      | 
      | for k = 1:length(blocks)
      |     if contains(extractAfter(blocks{k,1}, '/'), 'Source')
      |         set_param(blocks{k}, 'BackgroundColor', '[0.929000, 0.490000, 0.439000]');
      |     end
      | end
  Bus_25 : MATLAB Function  TreatAsAtomicUnit=on  mask{MyInitialization=0, Bus_ID=25, Fault_flag=1}
      mask prompts: Bus_ID "Bus ID"; Fault_flag "Fault flag"
      settings: CopyFcn=|
      | Component_Name = get_param(gcb, 'Name');
      | set_param(gcb, 'Bus_ID', num2str(strtrim(extractAfter(Component_Name, '_'))));
      | 
      | blocks = find_system(gcs, 'SearchDepth', 1, 'Type', 'Block');
      | 
      | for k = 1:length(blocks)
      |     if contains(extractAfter(blocks{k,1}, '/'), 'Source')
      |         set_param(blocks{k}, 'BackgroundColor', '[0.929000, 0.490000, 0.439000]');
      |     end
      | end
      settings: NameChangeFcn=|
      | Component_Name = get_param(gcb, 'Name');
      | old_ID = get_param(gcb, 'Bus_ID');
      | 
      | pattern = '_\d+';
      | match = regexp(Component_Name, pattern, 'match');
      | 
      | if ~isempty(match)
      |     if ~isequal(old_ID, num2str(strtrim(extractAfter(Component_Name, '_'))))
      |         set_param(gcb, 'Bus_ID', num2str(strtrim(extractAfter(Component_Name, '_'))));
      |     end
      | else
      |     newName = [Component_Name '_' old_ID];
      |     set_param(gcb, 'Name', newName);
      | end
      | 
      | if ~isequal(old_ID, get_param(gcb, 'Bus_ID'))
      | 
      |     data = get_param(gcb, 'PortConnectivity');
      |     for i = 1:numel(data)
      |         sourceHandle = data(i,1).SrcBlock;
      |         if ~isempty(sourceHandle) && sourceHandle ~= -1
      |             sourceParams = get_param(sourceHandle, 'DialogParameters');
      |             fn = fieldnames(sourceParams);
      |             if contains(fn{2}, 'Source')
      |                 Bus_ID = get_param(gcb, 'Bus_ID');
      |                 set_param(sourceHandle, 'Source_ID', Bus_ID);
      |             end
      |         end
      |     end
      | 
      |     blocks = find_system(gcs, 'SearchDepth', 1, 'Type', 'Block');
      | 
      |     for k = 1:length(blocks)
      |         if contains(extractAfter(blocks{k,1}, '/'), 'Source')
      |             set_param(blocks{k}, 'BackgroundColor', '[0.929000, 0.490000, 0.439000]');
      |         end
      |     end
      | 
      | end
      settings: PreDeleteFcn=|
      | blocks = find_system(gcs, 'SearchDepth', 1, 'Type', 'Block');
      | 
      | for k = 1:length(blocks)
      |     if contains(extractAfter(blocks{k,1}, '/'), 'Source')
      |         set_param(blocks{k}, 'BackgroundColor', '[0.929000, 0.490000, 0.439000]');
      |     end
      | end
  Bus_26 : MATLAB Function  TreatAsAtomicUnit=on  mask{MyInitialization=0, Bus_ID=26, Fault_flag=1}
      mask prompts: Bus_ID "Bus ID"; Fault_flag "Fault flag"
      settings: CopyFcn=|
      | Component_Name = get_param(gcb, 'Name');
      | set_param(gcb, 'Bus_ID', num2str(strtrim(extractAfter(Component_Name, '_'))));
      | 
      | blocks = find_system(gcs, 'SearchDepth', 1, 'Type', 'Block');
      | 
      | for k = 1:length(blocks)
      |     if contains(extractAfter(blocks{k,1}, '/'), 'Source')
      |         set_param(blocks{k}, 'BackgroundColor', '[0.929000, 0.490000, 0.439000]');
      |     end
      | end
      settings: NameChangeFcn=|
      | Component_Name = get_param(gcb, 'Name');
      | old_ID = get_param(gcb, 'Bus_ID');
      | 
      | pattern = '_\d+';
      | match = regexp(Component_Name, pattern, 'match');
      | 
      | if ~isempty(match)
      |     if ~isequal(old_ID, num2str(strtrim(extractAfter(Component_Name, '_'))))
      |         set_param(gcb, 'Bus_ID', num2str(strtrim(extractAfter(Component_Name, '_'))));
      |     end
      | else
      |     newName = [Component_Name '_' old_ID];
      |     set_param(gcb, 'Name', newName);
      | end
      | 
      | if ~isequal(old_ID, get_param(gcb, 'Bus_ID'))
      | 
      |     data = get_param(gcb, 'PortConnectivity');
      |     for i = 1:numel(data)
      |         sourceHandle = data(i,1).SrcBlock;
      |         if ~isempty(sourceHandle) && sourceHandle ~= -1
      |             sourceParams = get_param(sourceHandle, 'DialogParameters');
      |             fn = fieldnames(sourceParams);
      |             if contains(fn{2}, 'Source')
      |                 Bus_ID = get_param(gcb, 'Bus_ID');
      |                 set_param(sourceHandle, 'Source_ID', Bus_ID);
      |             end
      |         end
      |     end
      | 
      |     blocks = find_system(gcs, 'SearchDepth', 1, 'Type', 'Block');
      | 
      |     for k = 1:length(blocks)
      |         if contains(extractAfter(blocks{k,1}, '/'), 'Source')
      |             set_param(blocks{k}, 'BackgroundColor', '[0.929000, 0.490000, 0.439000]');
      |         end
      |     end
      | 
      | end
      settings: PreDeleteFcn=|
      | blocks = find_system(gcs, 'SearchDepth', 1, 'Type', 'Block');
      | 
      | for k = 1:length(blocks)
      |     if contains(extractAfter(blocks{k,1}, '/'), 'Source')
      |         set_param(blocks{k}, 'BackgroundColor', '[0.929000, 0.490000, 0.439000]');
      |     end
      | end
  Bus_27 : MATLAB Function  TreatAsAtomicUnit=on  mask{MyInitialization=0, Bus_ID=27, Fault_flag=1}
      mask prompts: Bus_ID "Bus ID"; Fault_flag "Fault flag"
      settings: CopyFcn=|
      | Component_Name = get_param(gcb, 'Name');
      | set_param(gcb, 'Bus_ID', num2str(strtrim(extractAfter(Component_Name, '_'))));
      | 
      | blocks = find_system(gcs, 'SearchDepth', 1, 'Type', 'Block');
      | 
      | for k = 1:length(blocks)
      |     if contains(extractAfter(blocks{k,1}, '/'), 'Source')
      |         set_param(blocks{k}, 'BackgroundColor', '[0.929000, 0.490000, 0.439000]');
      |     end
      | end
      settings: NameChangeFcn=|
      | Component_Name = get_param(gcb, 'Name');
      | old_ID = get_param(gcb, 'Bus_ID');
      | 
      | pattern = '_\d+';
      | match = regexp(Component_Name, pattern, 'match');
      | 
      | if ~isempty(match)
      |     if ~isequal(old_ID, num2str(strtrim(extractAfter(Component_Name, '_'))))
      |         set_param(gcb, 'Bus_ID', num2str(strtrim(extractAfter(Component_Name, '_'))));
      |     end
      | else
      |     newName = [Component_Name '_' old_ID];
      |     set_param(gcb, 'Name', newName);
      | end
      | 
      | if ~isequal(old_ID, get_param(gcb, 'Bus_ID'))
      | 
      |     data = get_param(gcb, 'PortConnectivity');
      |     for i = 1:numel(data)
      |         sourceHandle = data(i,1).SrcBlock;
      |         if ~isempty(sourceHandle) && sourceHandle ~= -1
      |             sourceParams = get_param(sourceHandle, 'DialogParameters');
      |             fn = fieldnames(sourceParams);
      |             if contains(fn{2}, 'Source')
      |                 Bus_ID = get_param(gcb, 'Bus_ID');
      |                 set_param(sourceHandle, 'Source_ID', Bus_ID);
      |             end
      |         end
      |     end
      | 
      |     blocks = find_system(gcs, 'SearchDepth', 1, 'Type', 'Block');
      | 
      |     for k = 1:length(blocks)
      |         if contains(extractAfter(blocks{k,1}, '/'), 'Source')
      |             set_param(blocks{k}, 'BackgroundColor', '[0.929000, 0.490000, 0.439000]');
      |         end
      |     end
      | 
      | end
      settings: PreDeleteFcn=|
      | blocks = find_system(gcs, 'SearchDepth', 1, 'Type', 'Block');
      | 
      | for k = 1:length(blocks)
      |     if contains(extractAfter(blocks{k,1}, '/'), 'Source')
      |         set_param(blocks{k}, 'BackgroundColor', '[0.929000, 0.490000, 0.439000]');
      |     end
      | end
  Bus_28 : MATLAB Function  TreatAsAtomicUnit=on  mask{MyInitialization=0, Bus_ID=28, Fault_flag=1}
      mask prompts: Bus_ID "Bus ID"; Fault_flag "Fault flag"
      settings: CopyFcn=|
      | Component_Name = get_param(gcb, 'Name');
      | set_param(gcb, 'Bus_ID', num2str(strtrim(extractAfter(Component_Name, '_'))));
      | 
      | blocks = find_system(gcs, 'SearchDepth', 1, 'Type', 'Block');
      | 
      | for k = 1:length(blocks)
      |     if contains(extractAfter(blocks{k,1}, '/'), 'Source')
      |         set_param(blocks{k}, 'BackgroundColor', '[0.929000, 0.490000, 0.439000]');
      |     end
      | end
      settings: NameChangeFcn=|
      | Component_Name = get_param(gcb, 'Name');
      | old_ID = get_param(gcb, 'Bus_ID');
      | 
      | pattern = '_\d+';
      | match = regexp(Component_Name, pattern, 'match');
      | 
      | if ~isempty(match)
      |     if ~isequal(old_ID, num2str(strtrim(extractAfter(Component_Name, '_'))))
      |         set_param(gcb, 'Bus_ID', num2str(strtrim(extractAfter(Component_Name, '_'))));
      |     end
      | else
      |     newName = [Component_Name '_' old_ID];
      |     set_param(gcb, 'Name', newName);
      | end
      | 
      | if ~isequal(old_ID, get_param(gcb, 'Bus_ID'))
      | 
      |     data = get_param(gcb, 'PortConnectivity');
      |     for i = 1:numel(data)
      |         sourceHandle = data(i,1).SrcBlock;
      |         if ~isempty(sourceHandle) && sourceHandle ~= -1
      |             sourceParams = get_param(sourceHandle, 'DialogParameters');
      |             fn = fieldnames(sourceParams);
      |             if contains(fn{2}, 'Source')
      |                 Bus_ID = get_param(gcb, 'Bus_ID');
      |                 set_param(sourceHandle, 'Source_ID', Bus_ID);
      |             end
      |         end
      |     end
      | 
      |     blocks = find_system(gcs, 'SearchDepth', 1, 'Type', 'Block');
      | 
      |     for k = 1:length(blocks)
      |         if contains(extractAfter(blocks{k,1}, '/'), 'Source')
      |             set_param(blocks{k}, 'BackgroundColor', '[0.929000, 0.490000, 0.439000]');
      |         end
      |     end
      | 
      | end
      settings: PreDeleteFcn=|
      | blocks = find_system(gcs, 'SearchDepth', 1, 'Type', 'Block');
      | 
      | for k = 1:length(blocks)
      |     if contains(extractAfter(blocks{k,1}, '/'), 'Source')
      |         set_param(blocks{k}, 'BackgroundColor', '[0.929000, 0.490000, 0.439000]');
      |     end
      | end
  Bus_29 : MATLAB Function  TreatAsAtomicUnit=on  mask{MyInitialization=0, Bus_ID=29, Fault_flag=1}
      mask prompts: Bus_ID "Bus ID"; Fault_flag "Fault flag"
      settings: CopyFcn=|
      | Component_Name = get_param(gcb, 'Name');
      | set_param(gcb, 'Bus_ID', num2str(strtrim(extractAfter(Component_Name, '_'))));
      | 
      | blocks = find_system(gcs, 'SearchDepth', 1, 'Type', 'Block');
      | 
      | for k = 1:length(blocks)
      |     if contains(extractAfter(blocks{k,1}, '/'), 'Source')
      |         set_param(blocks{k}, 'BackgroundColor', '[0.929000, 0.490000, 0.439000]');
      |     end
      | end
      settings: NameChangeFcn=|
      | Component_Name = get_param(gcb, 'Name');
      | old_ID = get_param(gcb, 'Bus_ID');
      | 
      | pattern = '_\d+';
      | match = regexp(Component_Name, pattern, 'match');
      | 
      | if ~isempty(match)
      |     if ~isequal(old_ID, num2str(strtrim(extractAfter(Component_Name, '_'))))
      |         set_param(gcb, 'Bus_ID', num2str(strtrim(extractAfter(Component_Name, '_'))));
      |     end
      | else
      |     newName = [Component_Name '_' old_ID];
      |     set_param(gcb, 'Name', newName);
      | end
      | 
      | if ~isequal(old_ID, get_param(gcb, 'Bus_ID'))
      | 
      |     data = get_param(gcb, 'PortConnectivity');
      |     for i = 1:numel(data)
      |         sourceHandle = data(i,1).SrcBlock;
      |         if ~isempty(sourceHandle) && sourceHandle ~= -1
      |             sourceParams = get_param(sourceHandle, 'DialogParameters');
      |             fn = fieldnames(sourceParams);
      |             if contains(fn{2}, 'Source')
      |                 Bus_ID = get_param(gcb, 'Bus_ID');
      |                 set_param(sourceHandle, 'Source_ID', Bus_ID);
      |             end
      |         end
      |     end
      | 
      |     blocks = find_system(gcs, 'SearchDepth', 1, 'Type', 'Block');
      | 
      |     for k = 1:length(blocks)
      |         if contains(extractAfter(blocks{k,1}, '/'), 'Source')
      |             set_param(blocks{k}, 'BackgroundColor', '[0.929000, 0.490000, 0.439000]');
      |         end
      |     end
      | 
      | end
      settings: PreDeleteFcn=|
      | blocks = find_system(gcs, 'SearchDepth', 1, 'Type', 'Block');
      | 
      | for k = 1:length(blocks)
      |     if contains(extractAfter(blocks{k,1}, '/'), 'Source')
      |         set_param(blocks{k}, 'BackgroundColor', '[0.929000, 0.490000, 0.439000]');
      |     end
      | end
  Bus_3 : MATLAB Function  TreatAsAtomicUnit=on  mask{MyInitialization=0, Bus_ID=3, Fault_flag=1}
      mask prompts: Bus_ID "Bus ID"; Fault_flag "Fault flag"
      settings: CopyFcn=|
      | Component_Name = get_param(gcb, 'Name');
      | set_param(gcb, 'Bus_ID', num2str(strtrim(extractAfter(Component_Name, '_'))));
      | 
      | blocks = find_system(gcs, 'SearchDepth', 1, 'Type', 'Block');
      | 
      | for k = 1:length(blocks)
      |     if contains(extractAfter(blocks{k,1}, '/'), 'Source')
      |         set_param(blocks{k}, 'BackgroundColor', '[0.929000, 0.490000, 0.439000]');
      |     end
      | end
      settings: NameChangeFcn=|
      | Component_Name = get_param(gcb, 'Name');
      | old_ID = get_param(gcb, 'Bus_ID');
      | 
      | pattern = '_\d+';
      | match = regexp(Component_Name, pattern, 'match');
      | 
      | if ~isempty(match)
      |     if ~isequal(old_ID, num2str(strtrim(extractAfter(Component_Name, '_'))))
      |         set_param(gcb, 'Bus_ID', num2str(strtrim(extractAfter(Component_Name, '_'))));
      |     end
      | else
      |     newName = [Component_Name '_' old_ID];
      |     set_param(gcb, 'Name', newName);
      | end
      | 
      | if ~isequal(old_ID, get_param(gcb, 'Bus_ID'))
      | 
      |     data = get_param(gcb, 'PortConnectivity');
      |     for i = 1:numel(data)
      |         sourceHandle = data(i,1).SrcBlock;
      |         if ~isempty(sourceHandle) && sourceHandle ~= -1
      |             sourceParams = get_param(sourceHandle, 'DialogParameters');
      |             fn = fieldnames(sourceParams);
      |             if contains(fn{2}, 'Source')
      |                 Bus_ID = get_param(gcb, 'Bus_ID');
      |                 set_param(sourceHandle, 'Source_ID', Bus_ID);
      |             end
      |         end
      |     end
      | 
      |     blocks = find_system(gcs, 'SearchDepth', 1, 'Type', 'Block');
      | 
      |     for k = 1:length(blocks)
      |         if contains(extractAfter(blocks{k,1}, '/'), 'Source')
      |             set_param(blocks{k}, 'BackgroundColor', '[0.929000, 0.490000, 0.439000]');
      |         end
      |     end
      | 
      | end
      settings: PreDeleteFcn=|
      | blocks = find_system(gcs, 'SearchDepth', 1, 'Type', 'Block');
      | 
      | for k = 1:length(blocks)
      |     if contains(extractAfter(blocks{k,1}, '/'), 'Source')
      |         set_param(blocks{k}, 'BackgroundColor', '[0.929000, 0.490000, 0.439000]');
      |     end
      | end
  Bus_30 : MATLAB Function  TreatAsAtomicUnit=on  mask{MyInitialization=0, Bus_ID=30, Fault_flag=1}
      mask prompts: Bus_ID "Bus ID"; Fault_flag "Fault flag"
      settings: CopyFcn=|
      | Component_Name = get_param(gcb, 'Name');
      | set_param(gcb, 'Bus_ID', num2str(strtrim(extractAfter(Component_Name, '_'))));
      | 
      | blocks = find_system(gcs, 'SearchDepth', 1, 'Type', 'Block');
      | 
      | for k = 1:length(blocks)
      |     if contains(extractAfter(blocks{k,1}, '/'), 'Source')
      |         set_param(blocks{k}, 'BackgroundColor', '[0.929000, 0.490000, 0.439000]');
      |     end
      | end
      settings: NameChangeFcn=|
      | Component_Name = get_param(gcb, 'Name');
      | old_ID = get_param(gcb, 'Bus_ID');
      | 
      | pattern = '_\d+';
      | match = regexp(Component_Name, pattern, 'match');
      | 
      | if ~isempty(match)
      |     if ~isequal(old_ID, num2str(strtrim(extractAfter(Component_Name, '_'))))
      |         set_param(gcb, 'Bus_ID', num2str(strtrim(extractAfter(Component_Name, '_'))));
      |     end
      | else
      |     newName = [Component_Name '_' old_ID];
      |     set_param(gcb, 'Name', newName);
      | end
      | 
      | if ~isequal(old_ID, get_param(gcb, 'Bus_ID'))
      | 
      |     data = get_param(gcb, 'PortConnectivity');
      |     for i = 1:numel(data)
      |         sourceHandle = data(i,1).SrcBlock;
      |         if ~isempty(sourceHandle) && sourceHandle ~= -1
      |             sourceParams = get_param(sourceHandle, 'DialogParameters');
      |             fn = fieldnames(sourceParams);
      |             if contains(fn{2}, 'Source')
      |                 Bus_ID = get_param(gcb, 'Bus_ID');
      |                 set_param(sourceHandle, 'Source_ID', Bus_ID);
      |             end
      |         end
      |     end
      | 
      |     blocks = find_system(gcs, 'SearchDepth', 1, 'Type', 'Block');
      | 
      |     for k = 1:length(blocks)
      |         if contains(extractAfter(blocks{k,1}, '/'), 'Source')
      |             set_param(blocks{k}, 'BackgroundColor', '[0.929000, 0.490000, 0.439000]');
      |         end
      |     end
      | 
      | end
      settings: PreDeleteFcn=|
      | blocks = find_system(gcs, 'SearchDepth', 1, 'Type', 'Block');
      | 
      | for k = 1:length(blocks)
      |     if contains(extractAfter(blocks{k,1}, '/'), 'Source')
      |         set_param(blocks{k}, 'BackgroundColor', '[0.929000, 0.490000, 0.439000]');
      |     end
      | end
  Bus_31 : MATLAB Function  TreatAsAtomicUnit=on  mask{MyInitialization=0, Bus_ID=31, Fault_flag=1}
      mask prompts: Bus_ID "Bus ID"; Fault_flag "Fault flag"
      settings: CopyFcn=|
      | Component_Name = get_param(gcb, 'Name');
      | set_param(gcb, 'Bus_ID', num2str(strtrim(extractAfter(Component_Name, '_'))));
      | 
      | blocks = find_system(gcs, 'SearchDepth', 1, 'Type', 'Block');
      | 
      | for k = 1:length(blocks)
      |     if contains(extractAfter(blocks{k,1}, '/'), 'Source')
      |         set_param(blocks{k}, 'BackgroundColor', '[0.929000, 0.490000, 0.439000]');
      |     end
      | end
      settings: NameChangeFcn=|
      | Component_Name = get_param(gcb, 'Name');
      | old_ID = get_param(gcb, 'Bus_ID');
      | 
      | pattern = '_\d+';
      | match = regexp(Component_Name, pattern, 'match');
      | 
      | if ~isempty(match)
      |     if ~isequal(old_ID, num2str(strtrim(extractAfter(Component_Name, '_'))))
      |         set_param(gcb, 'Bus_ID', num2str(strtrim(extractAfter(Component_Name, '_'))));
      |     end
      | else
      |     newName = [Component_Name '_' old_ID];
      |     set_param(gcb, 'Name', newName);
      | end
      | 
      | if ~isequal(old_ID, get_param(gcb, 'Bus_ID'))
      | 
      |     data = get_param(gcb, 'PortConnectivity');
      |     for i = 1:numel(data)
      |         sourceHandle = data(i,1).SrcBlock;
      |         if ~isempty(sourceHandle) && sourceHandle ~= -1
      |             sourceParams = get_param(sourceHandle, 'DialogParameters');
      |             fn = fieldnames(sourceParams);
      |             if contains(fn{2}, 'Source')
      |                 Bus_ID = get_param(gcb, 'Bus_ID');
      |                 set_param(sourceHandle, 'Source_ID', Bus_ID);
      |             end
      |         end
      |     end
      | 
      |     blocks = find_system(gcs, 'SearchDepth', 1, 'Type', 'Block');
      | 
      |     for k = 1:length(blocks)
      |         if contains(extractAfter(blocks{k,1}, '/'), 'Source')
      |             set_param(blocks{k}, 'BackgroundColor', '[0.929000, 0.490000, 0.439000]');
      |         end
      |     end
      | 
      | end
      settings: PreDeleteFcn=|
      | blocks = find_system(gcs, 'SearchDepth', 1, 'Type', 'Block');
      | 
      | for k = 1:length(blocks)
      |     if contains(extractAfter(blocks{k,1}, '/'), 'Source')
      |         set_param(blocks{k}, 'BackgroundColor', '[0.929000, 0.490000, 0.439000]');
      |     end
      | end
  Bus_32 : MATLAB Function  TreatAsAtomicUnit=on  mask{MyInitialization=0, Bus_ID=32, Fault_flag=1}
      mask prompts: Bus_ID "Bus ID"; Fault_flag "Fault flag"
      settings: CopyFcn=|
      | Component_Name = get_param(gcb, 'Name');
      | set_param(gcb, 'Bus_ID', num2str(strtrim(extractAfter(Component_Name, '_'))));
      | 
      | blocks = find_system(gcs, 'SearchDepth', 1, 'Type', 'Block');
      | 
      | for k = 1:length(blocks)
      |     if contains(extractAfter(blocks{k,1}, '/'), 'Source')
      |         set_param(blocks{k}, 'BackgroundColor', '[0.929000, 0.490000, 0.439000]');
      |     end
      | end
      settings: NameChangeFcn=|
      | Component_Name = get_param(gcb, 'Name');
      | old_ID = get_param(gcb, 'Bus_ID');
      | 
      | pattern = '_\d+';
      | match = regexp(Component_Name, pattern, 'match');
      | 
      | if ~isempty(match)
      |     if ~isequal(old_ID, num2str(strtrim(extractAfter(Component_Name, '_'))))
      |         set_param(gcb, 'Bus_ID', num2str(strtrim(extractAfter(Component_Name, '_'))));
      |     end
      | else
      |     newName = [Component_Name '_' old_ID];
      |     set_param(gcb, 'Name', newName);
      | end
      | 
      | if ~isequal(old_ID, get_param(gcb, 'Bus_ID'))
      | 
      |     data = get_param(gcb, 'PortConnectivity');
      |     for i = 1:numel(data)
      |         sourceHandle = data(i,1).SrcBlock;
      |         if ~isempty(sourceHandle) && sourceHandle ~= -1
      |             sourceParams = get_param(sourceHandle, 'DialogParameters');
      |             fn = fieldnames(sourceParams);
      |             if contains(fn{2}, 'Source')
      |                 Bus_ID = get_param(gcb, 'Bus_ID');
      |                 set_param(sourceHandle, 'Source_ID', Bus_ID);
      |             end
      |         end
      |     end
      | 
      |     blocks = find_system(gcs, 'SearchDepth', 1, 'Type', 'Block');
      | 
      |     for k = 1:length(blocks)
      |         if contains(extractAfter(blocks{k,1}, '/'), 'Source')
      |             set_param(blocks{k}, 'BackgroundColor', '[0.929000, 0.490000, 0.439000]');
      |         end
      |     end
      | 
      | end
      settings: PreDeleteFcn=|
      | blocks = find_system(gcs, 'SearchDepth', 1, 'Type', 'Block');
      | 
      | for k = 1:length(blocks)
      |     if contains(extractAfter(blocks{k,1}, '/'), 'Source')
      |         set_param(blocks{k}, 'BackgroundColor', '[0.929000, 0.490000, 0.439000]');
      |     end
      | end
  Bus_33 : MATLAB Function  TreatAsAtomicUnit=on  mask{MyInitialization=0, Bus_ID=33, Fault_flag=1}
      mask prompts: Bus_ID "Bus ID"; Fault_flag "Fault flag"
      settings: CopyFcn=|
      | Component_Name = get_param(gcb, 'Name');
      | set_param(gcb, 'Bus_ID', num2str(strtrim(extractAfter(Component_Name, '_'))));
      | 
      | blocks = find_system(gcs, 'SearchDepth', 1, 'Type', 'Block');
      | 
      | for k = 1:length(blocks)
      |     if contains(extractAfter(blocks{k,1}, '/'), 'Source')
      |         set_param(blocks{k}, 'BackgroundColor', '[0.929000, 0.490000, 0.439000]');
      |     end
      | end
      settings: NameChangeFcn=|
      | Component_Name = get_param(gcb, 'Name');
      | old_ID = get_param(gcb, 'Bus_ID');
      | 
      | pattern = '_\d+';
      | match = regexp(Component_Name, pattern, 'match');
      | 
      | if ~isempty(match)
      |     if ~isequal(old_ID, num2str(strtrim(extractAfter(Component_Name, '_'))))
      |         set_param(gcb, 'Bus_ID', num2str(strtrim(extractAfter(Component_Name, '_'))));
      |     end
      | else
      |     newName = [Component_Name '_' old_ID];
      |     set_param(gcb, 'Name', newName);
      | end
      | 
      | if ~isequal(old_ID, get_param(gcb, 'Bus_ID'))
      | 
      |     data = get_param(gcb, 'PortConnectivity');
      |     for i = 1:numel(data)
      |         sourceHandle = data(i,1).SrcBlock;
      |         if ~isempty(sourceHandle) && sourceHandle ~= -1
      |             sourceParams = get_param(sourceHandle, 'DialogParameters');
      |             fn = fieldnames(sourceParams);
      |             if contains(fn{2}, 'Source')
      |                 Bus_ID = get_param(gcb, 'Bus_ID');
      |                 set_param(sourceHandle, 'Source_ID', Bus_ID);
      |             end
      |         end
      |     end
      | 
      |     blocks = find_system(gcs, 'SearchDepth', 1, 'Type', 'Block');
      | 
      |     for k = 1:length(blocks)
      |         if contains(extractAfter(blocks{k,1}, '/'), 'Source')
      |             set_param(blocks{k}, 'BackgroundColor', '[0.929000, 0.490000, 0.439000]');
      |         end
      |     end
      | 
      | end
      settings: PreDeleteFcn=|
      | blocks = find_system(gcs, 'SearchDepth', 1, 'Type', 'Block');
      | 
      | for k = 1:length(blocks)
      |     if contains(extractAfter(blocks{k,1}, '/'), 'Source')
      |         set_param(blocks{k}, 'BackgroundColor', '[0.929000, 0.490000, 0.439000]');
      |     end
      | end
  Bus_34 : MATLAB Function  TreatAsAtomicUnit=on  mask{MyInitialization=0, Bus_ID=34, Fault_flag=1}
      mask prompts: Bus_ID "Bus ID"; Fault_flag "Fault flag"
      settings: CopyFcn=|
      | Component_Name = get_param(gcb, 'Name');
      | set_param(gcb, 'Bus_ID', num2str(strtrim(extractAfter(Component_Name, '_'))));
      | 
      | blocks = find_system(gcs, 'SearchDepth', 1, 'Type', 'Block');
      | 
      | for k = 1:length(blocks)
      |     if contains(extractAfter(blocks{k,1}, '/'), 'Source')
      |         set_param(blocks{k}, 'BackgroundColor', '[0.929000, 0.490000, 0.439000]');
      |     end
      | end
      settings: NameChangeFcn=|
      | Component_Name = get_param(gcb, 'Name');
      | old_ID = get_param(gcb, 'Bus_ID');
      | 
      | pattern = '_\d+';
      | match = regexp(Component_Name, pattern, 'match');
      | 
      | if ~isempty(match)
      |     if ~isequal(old_ID, num2str(strtrim(extractAfter(Component_Name, '_'))))
      |         set_param(gcb, 'Bus_ID', num2str(strtrim(extractAfter(Component_Name, '_'))));
      |     end
      | else
      |     newName = [Component_Name '_' old_ID];
      |     set_param(gcb, 'Name', newName);
      | end
      | 
      | if ~isequal(old_ID, get_param(gcb, 'Bus_ID'))
      | 
      |     data = get_param(gcb, 'PortConnectivity');
      |     for i = 1:numel(data)
      |         sourceHandle = data(i,1).SrcBlock;
      |         if ~isempty(sourceHandle) && sourceHandle ~= -1
      |             sourceParams = get_param(sourceHandle, 'DialogParameters');
      |             fn = fieldnames(sourceParams);
      |             if contains(fn{2}, 'Source')
      |                 Bus_ID = get_param(gcb, 'Bus_ID');
      |                 set_param(sourceHandle, 'Source_ID', Bus_ID);
      |             end
      |         end
      |     end
      | 
      |     blocks = find_system(gcs, 'SearchDepth', 1, 'Type', 'Block');
      | 
      |     for k = 1:length(blocks)
      |         if contains(extractAfter(blocks{k,1}, '/'), 'Source')
      |             set_param(blocks{k}, 'BackgroundColor', '[0.929000, 0.490000, 0.439000]');
      |         end
      |     end
      | 
      | end
      settings: PreDeleteFcn=|
      | blocks = find_system(gcs, 'SearchDepth', 1, 'Type', 'Block');
      | 
      | for k = 1:length(blocks)
      |     if contains(extractAfter(blocks{k,1}, '/'), 'Source')
      |         set_param(blocks{k}, 'BackgroundColor', '[0.929000, 0.490000, 0.439000]');
      |     end
      | end
  Bus_35 : MATLAB Function  TreatAsAtomicUnit=on  mask{MyInitialization=0, Bus_ID=35, Fault_flag=1}
      mask prompts: Bus_ID "Bus ID"; Fault_flag "Fault flag"
      settings: CopyFcn=|
      | Component_Name = get_param(gcb, 'Name');
      | set_param(gcb, 'Bus_ID', num2str(strtrim(extractAfter(Component_Name, '_'))));
      | 
      | blocks = find_system(gcs, 'SearchDepth', 1, 'Type', 'Block');
      | 
      | for k = 1:length(blocks)
      |     if contains(extractAfter(blocks{k,1}, '/'), 'Source')
      |         set_param(blocks{k}, 'BackgroundColor', '[0.929000, 0.490000, 0.439000]');
      |     end
      | end
      settings: NameChangeFcn=|
      | Component_Name = get_param(gcb, 'Name');
      | old_ID = get_param(gcb, 'Bus_ID');
      | 
      | pattern = '_\d+';
      | match = regexp(Component_Name, pattern, 'match');
      | 
      | if ~isempty(match)
      |     if ~isequal(old_ID, num2str(strtrim(extractAfter(Component_Name, '_'))))
      |         set_param(gcb, 'Bus_ID', num2str(strtrim(extractAfter(Component_Name, '_'))));
      |     end
      | else
      |     newName = [Component_Name '_' old_ID];
      |     set_param(gcb, 'Name', newName);
      | end
      | 
      | if ~isequal(old_ID, get_param(gcb, 'Bus_ID'))
      | 
      |     data = get_param(gcb, 'PortConnectivity');
      |     for i = 1:numel(data)
      |         sourceHandle = data(i,1).SrcBlock;
      |         if ~isempty(sourceHandle) && sourceHandle ~= -1
      |             sourceParams = get_param(sourceHandle, 'DialogParameters');
      |             fn = fieldnames(sourceParams);
      |             if contains(fn{2}, 'Source')
      |                 Bus_ID = get_param(gcb, 'Bus_ID');
      |                 set_param(sourceHandle, 'Source_ID', Bus_ID);
      |             end
      |         end
      |     end
      | 
      |     blocks = find_system(gcs, 'SearchDepth', 1, 'Type', 'Block');
      | 
      |     for k = 1:length(blocks)
      |         if contains(extractAfter(blocks{k,1}, '/'), 'Source')
      |             set_param(blocks{k}, 'BackgroundColor', '[0.929000, 0.490000, 0.439000]');
      |         end
      |     end
      | 
      | end
      settings: PreDeleteFcn=|
      | blocks = find_system(gcs, 'SearchDepth', 1, 'Type', 'Block');
      | 
      | for k = 1:length(blocks)
      |     if contains(extractAfter(blocks{k,1}, '/'), 'Source')
      |         set_param(blocks{k}, 'BackgroundColor', '[0.929000, 0.490000, 0.439000]');
      |     end
      | end
  Bus_36 : MATLAB Function  TreatAsAtomicUnit=on  mask{MyInitialization=0, Bus_ID=36, Fault_flag=1}
      mask prompts: Bus_ID "Bus ID"; Fault_flag "Fault flag"
      settings: CopyFcn=|
      | Component_Name = get_param(gcb, 'Name');
      | set_param(gcb, 'Bus_ID', num2str(strtrim(extractAfter(Component_Name, '_'))));
      | 
      | blocks = find_system(gcs, 'SearchDepth', 1, 'Type', 'Block');
      | 
      | for k = 1:length(blocks)
      |     if contains(extractAfter(blocks{k,1}, '/'), 'Source')
      |         set_param(blocks{k}, 'BackgroundColor', '[0.929000, 0.490000, 0.439000]');
      |     end
      | end
      settings: NameChangeFcn=|
      | Component_Name = get_param(gcb, 'Name');
      | old_ID = get_param(gcb, 'Bus_ID');
      | 
      | pattern = '_\d+';
      | match = regexp(Component_Name, pattern, 'match');
      | 
      | if ~isempty(match)
      |     if ~isequal(old_ID, num2str(strtrim(extractAfter(Component_Name, '_'))))
      |         set_param(gcb, 'Bus_ID', num2str(strtrim(extractAfter(Component_Name, '_'))));
      |     end
      | else
      |     newName = [Component_Name '_' old_ID];
      |     set_param(gcb, 'Name', newName);
      | end
      | 
      | if ~isequal(old_ID, get_param(gcb, 'Bus_ID'))
      | 
      |     data = get_param(gcb, 'PortConnectivity');
      |     for i = 1:numel(data)
      |         sourceHandle = data(i,1).SrcBlock;
      |         if ~isempty(sourceHandle) && sourceHandle ~= -1
      |             sourceParams = get_param(sourceHandle, 'DialogParameters');
      |             fn = fieldnames(sourceParams);
      |             if contains(fn{2}, 'Source')
      |                 Bus_ID = get_param(gcb, 'Bus_ID');
      |                 set_param(sourceHandle, 'Source_ID', Bus_ID);
      |             end
      |         end
      |     end
      | 
      |     blocks = find_system(gcs, 'SearchDepth', 1, 'Type', 'Block');
      | 
      |     for k = 1:length(blocks)
      |         if contains(extractAfter(blocks{k,1}, '/'), 'Source')
      |             set_param(blocks{k}, 'BackgroundColor', '[0.929000, 0.490000, 0.439000]');
      |         end
      |     end
      | 
      | end
      settings: PreDeleteFcn=|
      | blocks = find_system(gcs, 'SearchDepth', 1, 'Type', 'Block');
      | 
      | for k = 1:length(blocks)
      |     if contains(extractAfter(blocks{k,1}, '/'), 'Source')
      |         set_param(blocks{k}, 'BackgroundColor', '[0.929000, 0.490000, 0.439000]');
      |     end
      | end
  Bus_37 : MATLAB Function  TreatAsAtomicUnit=on  mask{MyInitialization=0, Bus_ID=37, Fault_flag=1}
      mask prompts: Bus_ID "Bus ID"; Fault_flag "Fault flag"
      settings: CopyFcn=|
      | Component_Name = get_param(gcb, 'Name');
      | set_param(gcb, 'Bus_ID', num2str(strtrim(extractAfter(Component_Name, '_'))));
      | 
      | blocks = find_system(gcs, 'SearchDepth', 1, 'Type', 'Block');
      | 
      | for k = 1:length(blocks)
      |     if contains(extractAfter(blocks{k,1}, '/'), 'Source')
      |         set_param(blocks{k}, 'BackgroundColor', '[0.929000, 0.490000, 0.439000]');
      |     end
      | end
      settings: NameChangeFcn=|
      | Component_Name = get_param(gcb, 'Name');
      | old_ID = get_param(gcb, 'Bus_ID');
      | 
      | pattern = '_\d+';
      | match = regexp(Component_Name, pattern, 'match');
      | 
      | if ~isempty(match)
      |     if ~isequal(old_ID, num2str(strtrim(extractAfter(Component_Name, '_'))))
      |         set_param(gcb, 'Bus_ID', num2str(strtrim(extractAfter(Component_Name, '_'))));
      |     end
      | else
      |     newName = [Component_Name '_' old_ID];
      |     set_param(gcb, 'Name', newName);
      | end
      | 
      | if ~isequal(old_ID, get_param(gcb, 'Bus_ID'))
      | 
      |     data = get_param(gcb, 'PortConnectivity');
      |     for i = 1:numel(data)
      |         sourceHandle = data(i,1).SrcBlock;
      |         if ~isempty(sourceHandle) && sourceHandle ~= -1
      |             sourceParams = get_param(sourceHandle, 'DialogParameters');
      |             fn = fieldnames(sourceParams);
      |             if contains(fn{2}, 'Source')
      |                 Bus_ID = get_param(gcb, 'Bus_ID');
      |                 set_param(sourceHandle, 'Source_ID', Bus_ID);
      |             end
      |         end
      |     end
      | 
      |     blocks = find_system(gcs, 'SearchDepth', 1, 'Type', 'Block');
      | 
      |     for k = 1:length(blocks)
      |         if contains(extractAfter(blocks{k,1}, '/'), 'Source')
      |             set_param(blocks{k}, 'BackgroundColor', '[0.929000, 0.490000, 0.439000]');
      |         end
      |     end
      | 
      | end
      settings: PreDeleteFcn=|
      | blocks = find_system(gcs, 'SearchDepth', 1, 'Type', 'Block');
      | 
      | for k = 1:length(blocks)
      |     if contains(extractAfter(blocks{k,1}, '/'), 'Source')
      |         set_param(blocks{k}, 'BackgroundColor', '[0.929000, 0.490000, 0.439000]');
      |     end
      | end
  Bus_38 : MATLAB Function  TreatAsAtomicUnit=on  mask{MyInitialization=0, Bus_ID=38, Fault_flag=1}
      mask prompts: Bus_ID "Bus ID"; Fault_flag "Fault flag"
      settings: CopyFcn=|
      | Component_Name = get_param(gcb, 'Name');
      | set_param(gcb, 'Bus_ID', num2str(strtrim(extractAfter(Component_Name, '_'))));
      | 
      | blocks = find_system(gcs, 'SearchDepth', 1, 'Type', 'Block');
      | 
      | for k = 1:length(blocks)
      |     if contains(extractAfter(blocks{k,1}, '/'), 'Source')
      |         set_param(blocks{k}, 'BackgroundColor', '[0.929000, 0.490000, 0.439000]');
      |     end
      | end
      settings: NameChangeFcn=|
      | Component_Name = get_param(gcb, 'Name');
      | old_ID = get_param(gcb, 'Bus_ID');
      | 
      | pattern = '_\d+';
      | match = regexp(Component_Name, pattern, 'match');
      | 
      | if ~isempty(match)
      |     if ~isequal(old_ID, num2str(strtrim(extractAfter(Component_Name, '_'))))
      |         set_param(gcb, 'Bus_ID', num2str(strtrim(extractAfter(Component_Name, '_'))));
      |     end
      | else
      |     newName = [Component_Name '_' old_ID];
      |     set_param(gcb, 'Name', newName);
      | end
      | 
      | if ~isequal(old_ID, get_param(gcb, 'Bus_ID'))
      | 
      |     data = get_param(gcb, 'PortConnectivity');
      |     for i = 1:numel(data)
      |         sourceHandle = data(i,1).SrcBlock;
      |         if ~isempty(sourceHandle) && sourceHandle ~= -1
      |             sourceParams = get_param(sourceHandle, 'DialogParameters');
      |             fn = fieldnames(sourceParams);
      |             if contains(fn{2}, 'Source')
      |                 Bus_ID = get_param(gcb, 'Bus_ID');
      |                 set_param(sourceHandle, 'Source_ID', Bus_ID);
      |             end
      |         end
      |     end
      | 
      |     blocks = find_system(gcs, 'SearchDepth', 1, 'Type', 'Block');
      | 
      |     for k = 1:length(blocks)
      |         if contains(extractAfter(blocks{k,1}, '/'), 'Source')
      |             set_param(blocks{k}, 'BackgroundColor', '[0.929000, 0.490000, 0.439000]');
      |         end
      |     end
      | 
      | end
      settings: PreDeleteFcn=|
      | blocks = find_system(gcs, 'SearchDepth', 1, 'Type', 'Block');
      | 
      | for k = 1:length(blocks)
      |     if contains(extractAfter(blocks{k,1}, '/'), 'Source')
      |         set_param(blocks{k}, 'BackgroundColor', '[0.929000, 0.490000, 0.439000]');
      |     end
      | end
  Bus_39 : MATLAB Function  TreatAsAtomicUnit=on  mask{MyInitialization=0, Bus_ID=39, Fault_flag=1}
      mask prompts: Bus_ID "Bus ID"; Fault_flag "Fault flag"
      settings: CopyFcn=|
      | Component_Name = get_param(gcb, 'Name');
      | set_param(gcb, 'Bus_ID', num2str(strtrim(extractAfter(Component_Name, '_'))));
      | 
      | blocks = find_system(gcs, 'SearchDepth', 1, 'Type', 'Block');
      | 
      | for k = 1:length(blocks)
      |     if contains(extractAfter(blocks{k,1}, '/'), 'Source')
      |         set_param(blocks{k}, 'BackgroundColor', '[0.929000, 0.490000, 0.439000]');
      |     end
      | end
      settings: NameChangeFcn=|
      | Component_Name = get_param(gcb, 'Name');
      | old_ID = get_param(gcb, 'Bus_ID');
      | 
      | pattern = '_\d+';
      | match = regexp(Component_Name, pattern, 'match');
      | 
      | if ~isempty(match)
      |     if ~isequal(old_ID, num2str(strtrim(extractAfter(Component_Name, '_'))))
      |         set_param(gcb, 'Bus_ID', num2str(strtrim(extractAfter(Component_Name, '_'))));
      |     end
      | else
      |     newName = [Component_Name '_' old_ID];
      |     set_param(gcb, 'Name', newName);
      | end
      | 
      | if ~isequal(old_ID, get_param(gcb, 'Bus_ID'))
      | 
      |     data = get_param(gcb, 'PortConnectivity');
      |     for i = 1:numel(data)
      |         sourceHandle = data(i,1).SrcBlock;
      |         if ~isempty(sourceHandle) && sourceHandle ~= -1
      |             sourceParams = get_param(sourceHandle, 'DialogParameters');
      |             fn = fieldnames(sourceParams);
      |             if contains(fn{2}, 'Source')
      |                 Bus_ID = get_param(gcb, 'Bus_ID');
      |                 set_param(sourceHandle, 'Source_ID', Bus_ID);
      |             end
      |         end
      |     end
      | 
      |     blocks = find_system(gcs, 'SearchDepth', 1, 'Type', 'Block');
      | 
      |     for k = 1:length(blocks)
      |         if contains(extractAfter(blocks{k,1}, '/'), 'Source')
      |             set_param(blocks{k}, 'BackgroundColor', '[0.929000, 0.490000, 0.439000]');
      |         end
      |     end
      | 
      | end
      settings: PreDeleteFcn=|
      | blocks = find_system(gcs, 'SearchDepth', 1, 'Type', 'Block');
      | 
      | for k = 1:length(blocks)
      |     if contains(extractAfter(blocks{k,1}, '/'), 'Source')
      |         set_param(blocks{k}, 'BackgroundColor', '[0.929000, 0.490000, 0.439000]');
      |     end
      | end
  Bus_4 : MATLAB Function  TreatAsAtomicUnit=on  mask{MyInitialization=0, Bus_ID=4, Fault_flag=1}
      mask prompts: Bus_ID "Bus ID"; Fault_flag "Fault flag"
      settings: CopyFcn=|
      | Component_Name = get_param(gcb, 'Name');
      | set_param(gcb, 'Bus_ID', num2str(strtrim(extractAfter(Component_Name, '_'))));
      | 
      | blocks = find_system(gcs, 'SearchDepth', 1, 'Type', 'Block');
      | 
      | for k = 1:length(blocks)
      |     if contains(extractAfter(blocks{k,1}, '/'), 'Source')
      |         set_param(blocks{k}, 'BackgroundColor', '[0.929000, 0.490000, 0.439000]');
      |     end
      | end
      settings: NameChangeFcn=|
      | Component_Name = get_param(gcb, 'Name');
      | old_ID = get_param(gcb, 'Bus_ID');
      | 
      | pattern = '_\d+';
      | match = regexp(Component_Name, pattern, 'match');
      | 
      | if ~isempty(match)
      |     if ~isequal(old_ID, num2str(strtrim(extractAfter(Component_Name, '_'))))
      |         set_param(gcb, 'Bus_ID', num2str(strtrim(extractAfter(Component_Name, '_'))));
      |     end
      | else
      |     newName = [Component_Name '_' old_ID];
      |     set_param(gcb, 'Name', newName);
      | end
      | 
      | if ~isequal(old_ID, get_param(gcb, 'Bus_ID'))
      | 
      |     data = get_param(gcb, 'PortConnectivity');
      |     for i = 1:numel(data)
      |         sourceHandle = data(i,1).SrcBlock;
      |         if ~isempty(sourceHandle) && sourceHandle ~= -1
      |             sourceParams = get_param(sourceHandle, 'DialogParameters');
      |             fn = fieldnames(sourceParams);
      |             if contains(fn{2}, 'Source')
      |                 Bus_ID = get_param(gcb, 'Bus_ID');
      |                 set_param(sourceHandle, 'Source_ID', Bus_ID);
      |             end
      |         end
      |     end
      | 
      |     blocks = find_system(gcs, 'SearchDepth', 1, 'Type', 'Block');
      | 
      |     for k = 1:length(blocks)
      |         if contains(extractAfter(blocks{k,1}, '/'), 'Source')
      |             set_param(blocks{k}, 'BackgroundColor', '[0.929000, 0.490000, 0.439000]');
      |         end
      |     end
      | 
      | end
      settings: PreDeleteFcn=|
      | blocks = find_system(gcs, 'SearchDepth', 1, 'Type', 'Block');
      | 
      | for k = 1:length(blocks)
      |     if contains(extractAfter(blocks{k,1}, '/'), 'Source')
      |         set_param(blocks{k}, 'BackgroundColor', '[0.929000, 0.490000, 0.439000]');
      |     end
      | end
  Bus_40 : MATLAB Function  TreatAsAtomicUnit=on  mask{MyInitialization=0, Bus_ID=40, Fault_flag=1}
      mask prompts: Bus_ID "Bus ID"; Fault_flag "Fault flag"
      settings: CopyFcn=|
      | Component_Name = get_param(gcb, 'Name');
      | set_param(gcb, 'Bus_ID', num2str(strtrim(extractAfter(Component_Name, '_'))));
      | 
      | blocks = find_system(gcs, 'SearchDepth', 1, 'Type', 'Block');
      | 
      | for k = 1:length(blocks)
      |     if contains(extractAfter(blocks{k,1}, '/'), 'Source')
      |         set_param(blocks{k}, 'BackgroundColor', '[0.929000, 0.490000, 0.439000]');
      |     end
      | end
      settings: NameChangeFcn=|
      | Component_Name = get_param(gcb, 'Name');
      | old_ID = get_param(gcb, 'Bus_ID');
      | 
      | pattern = '_\d+';
      | match = regexp(Component_Name, pattern, 'match');
      | 
      | if ~isempty(match)
      |     if ~isequal(old_ID, num2str(strtrim(extractAfter(Component_Name, '_'))))
      |         set_param(gcb, 'Bus_ID', num2str(strtrim(extractAfter(Component_Name, '_'))));
      |     end
      | else
      |     newName = [Component_Name '_' old_ID];
      |     set_param(gcb, 'Name', newName);
      | end
      | 
      | if ~isequal(old_ID, get_param(gcb, 'Bus_ID'))
      | 
      |     data = get_param(gcb, 'PortConnectivity');
      |     for i = 1:numel(data)
      |         sourceHandle = data(i,1).SrcBlock;
      |         if ~isempty(sourceHandle) && sourceHandle ~= -1
      |             sourceParams = get_param(sourceHandle, 'DialogParameters');
      |             fn = fieldnames(sourceParams);
      |             if contains(fn{2}, 'Source')
      |                 Bus_ID = get_param(gcb, 'Bus_ID');
      |                 set_param(sourceHandle, 'Source_ID', Bus_ID);
      |             end
      |         end
      |     end
      | 
      |     blocks = find_system(gcs, 'SearchDepth', 1, 'Type', 'Block');
      | 
      |     for k = 1:length(blocks)
      |         if contains(extractAfter(blocks{k,1}, '/'), 'Source')
      |             set_param(blocks{k}, 'BackgroundColor', '[0.929000, 0.490000, 0.439000]');
      |         end
      |     end
      | 
      | end
      settings: PreDeleteFcn=|
      | blocks = find_system(gcs, 'SearchDepth', 1, 'Type', 'Block');
      | 
      | for k = 1:length(blocks)
      |     if contains(extractAfter(blocks{k,1}, '/'), 'Source')
      |         set_param(blocks{k}, 'BackgroundColor', '[0.929000, 0.490000, 0.439000]');
      |     end
      | end
  Bus_41 : MATLAB Function  TreatAsAtomicUnit=on  mask{MyInitialization=0, Bus_ID=41, Fault_flag=1}
      mask prompts: Bus_ID "Bus ID"; Fault_flag "Fault flag"
      settings: CopyFcn=|
      | Component_Name = get_param(gcb, 'Name');
      | set_param(gcb, 'Bus_ID', num2str(strtrim(extractAfter(Component_Name, '_'))));
      | 
      | blocks = find_system(gcs, 'SearchDepth', 1, 'Type', 'Block');
      | 
      | for k = 1:length(blocks)
      |     if contains(extractAfter(blocks{k,1}, '/'), 'Source')
      |         set_param(blocks{k}, 'BackgroundColor', '[0.929000, 0.490000, 0.439000]');
      |     end
      | end
      settings: NameChangeFcn=|
      | Component_Name = get_param(gcb, 'Name');
      | old_ID = get_param(gcb, 'Bus_ID');
      | 
      | pattern = '_\d+';
      | match = regexp(Component_Name, pattern, 'match');
      | 
      | if ~isempty(match)
      |     if ~isequal(old_ID, num2str(strtrim(extractAfter(Component_Name, '_'))))
      |         set_param(gcb, 'Bus_ID', num2str(strtrim(extractAfter(Component_Name, '_'))));
      |     end
      | else
      |     newName = [Component_Name '_' old_ID];
      |     set_param(gcb, 'Name', newName);
      | end
      | 
      | if ~isequal(old_ID, get_param(gcb, 'Bus_ID'))
      | 
      |     data = get_param(gcb, 'PortConnectivity');
      |     for i = 1:numel(data)
      |         sourceHandle = data(i,1).SrcBlock;
      |         if ~isempty(sourceHandle) && sourceHandle ~= -1
      |             sourceParams = get_param(sourceHandle, 'DialogParameters');
      |             fn = fieldnames(sourceParams);
      |             if contains(fn{2}, 'Source')
      |                 Bus_ID = get_param(gcb, 'Bus_ID');
      |                 set_param(sourceHandle, 'Source_ID', Bus_ID);
      |             end
      |         end
      |     end
      | 
      |     blocks = find_system(gcs, 'SearchDepth', 1, 'Type', 'Block');
      | 
      |     for k = 1:length(blocks)
      |         if contains(extractAfter(blocks{k,1}, '/'), 'Source')
      |             set_param(blocks{k}, 'BackgroundColor', '[0.929000, 0.490000, 0.439000]');
      |         end
      |     end
      | 
      | end
      settings: PreDeleteFcn=|
      | blocks = find_system(gcs, 'SearchDepth', 1, 'Type', 'Block');
      | 
      | for k = 1:length(blocks)
      |     if contains(extractAfter(blocks{k,1}, '/'), 'Source')
      |         set_param(blocks{k}, 'BackgroundColor', '[0.929000, 0.490000, 0.439000]');
      |     end
      | end
  Bus_42 : MATLAB Function  TreatAsAtomicUnit=on  mask{MyInitialization=0, Bus_ID=42, Fault_flag=0}
      mask prompts: Bus_ID "Bus ID"; Fault_flag "Fault flag"
      settings: CopyFcn=|
      | Component_Name = get_param(gcb, 'Name');
      | set_param(gcb, 'Bus_ID', num2str(strtrim(extractAfter(Component_Name, '_'))));
      | 
      | blocks = find_system(gcs, 'SearchDepth', 1, 'Type', 'Block');
      | 
      | for k = 1:length(blocks)
      |     if contains(extractAfter(blocks{k,1}, '/'), 'Source')
      |         set_param(blocks{k}, 'BackgroundColor', '[0.929000, 0.490000, 0.439000]');
      |     end
      | end
      settings: NameChangeFcn=|
      | Component_Name = get_param(gcb, 'Name');
      | old_ID = get_param(gcb, 'Bus_ID');
      | 
      | pattern = '_\d+';
      | match = regexp(Component_Name, pattern, 'match');
      | 
      | if ~isempty(match)
      |     if ~isequal(old_ID, num2str(strtrim(extractAfter(Component_Name, '_'))))
      |         set_param(gcb, 'Bus_ID', num2str(strtrim(extractAfter(Component_Name, '_'))));
      |     end
      | else
      |     newName = [Component_Name '_' old_ID];
      |     set_param(gcb, 'Name', newName);
      | end
      | 
      | if ~isequal(old_ID, get_param(gcb, 'Bus_ID'))
      | 
      |     data = get_param(gcb, 'PortConnectivity');
      |     for i = 1:numel(data)
      |         sourceHandle = data(i,1).SrcBlock;
      |         if ~isempty(sourceHandle) && sourceHandle ~= -1
      |             sourceParams = get_param(sourceHandle, 'DialogParameters');
      |             fn = fieldnames(sourceParams);
      |             if contains(fn{2}, 'Source')
      |                 Bus_ID = get_param(gcb, 'Bus_ID');
      |                 set_param(sourceHandle, 'Source_ID', Bus_ID);
      |             end
      |         end
      |     end
      | 
      |     blocks = find_system(gcs, 'SearchDepth', 1, 'Type', 'Block');
      | 
      |     for k = 1:length(blocks)
      |         if contains(extractAfter(blocks{k,1}, '/'), 'Source')
      |             set_param(blocks{k}, 'BackgroundColor', '[0.929000, 0.490000, 0.439000]');
      |         end
      |     end
      | 
      | end
      settings: PreDeleteFcn=|
      | blocks = find_system(gcs, 'SearchDepth', 1, 'Type', 'Block');
      | 
      | for k = 1:length(blocks)
      |     if contains(extractAfter(blocks{k,1}, '/'), 'Source')
      |         set_param(blocks{k}, 'BackgroundColor', '[0.929000, 0.490000, 0.439000]');
      |     end
      | end
  Bus_43 : MATLAB Function  TreatAsAtomicUnit=on  mask{MyInitialization=0, Bus_ID=43, Fault_flag=1}
      mask prompts: Bus_ID "Bus ID"; Fault_flag "Fault flag"
      settings: CopyFcn=|
      | Component_Name = get_param(gcb, 'Name');
      | set_param(gcb, 'Bus_ID', num2str(strtrim(extractAfter(Component_Name, '_'))));
      | 
      | blocks = find_system(gcs, 'SearchDepth', 1, 'Type', 'Block');
      | 
      | for k = 1:length(blocks)
      |     if contains(extractAfter(blocks{k,1}, '/'), 'Source')
      |         set_param(blocks{k}, 'BackgroundColor', '[0.929000, 0.490000, 0.439000]');
      |     end
      | end
      settings: NameChangeFcn=|
      | Component_Name = get_param(gcb, 'Name');
      | old_ID = get_param(gcb, 'Bus_ID');
      | 
      | pattern = '_\d+';
      | match = regexp(Component_Name, pattern, 'match');
      | 
      | if ~isempty(match)
      |     if ~isequal(old_ID, num2str(strtrim(extractAfter(Component_Name, '_'))))
      |         set_param(gcb, 'Bus_ID', num2str(strtrim(extractAfter(Component_Name, '_'))));
      |     end
      | else
      |     newName = [Component_Name '_' old_ID];
      |     set_param(gcb, 'Name', newName);
      | end
      | 
      | if ~isequal(old_ID, get_param(gcb, 'Bus_ID'))
      | 
      |     data = get_param(gcb, 'PortConnectivity');
      |     for i = 1:numel(data)
      |         sourceHandle = data(i,1).SrcBlock;
      |         if ~isempty(sourceHandle) && sourceHandle ~= -1
      |             sourceParams = get_param(sourceHandle, 'DialogParameters');
      |             fn = fieldnames(sourceParams);
      |             if contains(fn{2}, 'Source')
      |                 Bus_ID = get_param(gcb, 'Bus_ID');
      |                 set_param(sourceHandle, 'Source_ID', Bus_ID);
      |             end
      |         end
      |     end
      | 
      |     blocks = find_system(gcs, 'SearchDepth', 1, 'Type', 'Block');
      | 
      |     for k = 1:length(blocks)
      |         if contains(extractAfter(blocks{k,1}, '/'), 'Source')
      |             set_param(blocks{k}, 'BackgroundColor', '[0.929000, 0.490000, 0.439000]');
      |         end
      |     end
      | 
      | end
      settings: PreDeleteFcn=|
      | blocks = find_system(gcs, 'SearchDepth', 1, 'Type', 'Block');
      | 
      | for k = 1:length(blocks)
      |     if contains(extractAfter(blocks{k,1}, '/'), 'Source')
      |         set_param(blocks{k}, 'BackgroundColor', '[0.929000, 0.490000, 0.439000]');
      |     end
      | end
  Bus_44 : MATLAB Function  TreatAsAtomicUnit=on  mask{MyInitialization=0, Bus_ID=44, Fault_flag=1}
      mask prompts: Bus_ID "Bus ID"; Fault_flag "Fault flag"
      settings: CopyFcn=|
      | Component_Name = get_param(gcb, 'Name');
      | set_param(gcb, 'Bus_ID', num2str(strtrim(extractAfter(Component_Name, '_'))));
      | 
      | blocks = find_system(gcs, 'SearchDepth', 1, 'Type', 'Block');
      | 
      | for k = 1:length(blocks)
      |     if contains(extractAfter(blocks{k,1}, '/'), 'Source')
      |         set_param(blocks{k}, 'BackgroundColor', '[0.929000, 0.490000, 0.439000]');
      |     end
      | end
      settings: NameChangeFcn=|
      | Component_Name = get_param(gcb, 'Name');
      | old_ID = get_param(gcb, 'Bus_ID');
      | 
      | pattern = '_\d+';
      | match = regexp(Component_Name, pattern, 'match');
      | 
      | if ~isempty(match)
      |     if ~isequal(old_ID, num2str(strtrim(extractAfter(Component_Name, '_'))))
      |         set_param(gcb, 'Bus_ID', num2str(strtrim(extractAfter(Component_Name, '_'))));
      |     end
      | else
      |     newName = [Component_Name '_' old_ID];
      |     set_param(gcb, 'Name', newName);
      | end
      | 
      | if ~isequal(old_ID, get_param(gcb, 'Bus_ID'))
      | 
      |     data = get_param(gcb, 'PortConnectivity');
      |     for i = 1:numel(data)
      |         sourceHandle = data(i,1).SrcBlock;
      |         if ~isempty(sourceHandle) && sourceHandle ~= -1
      |             sourceParams = get_param(sourceHandle, 'DialogParameters');
      |             fn = fieldnames(sourceParams);
      |             if contains(fn{2}, 'Source')
      |                 Bus_ID = get_param(gcb, 'Bus_ID');
      |                 set_param(sourceHandle, 'Source_ID', Bus_ID);
      |             end
      |         end
      |     end
      | 
      |     blocks = find_system(gcs, 'SearchDepth', 1, 'Type', 'Block');
      | 
      |     for k = 1:length(blocks)
      |         if contains(extractAfter(blocks{k,1}, '/'), 'Source')
      |             set_param(blocks{k}, 'BackgroundColor', '[0.929000, 0.490000, 0.439000]');
      |         end
      |     end
      | 
      | end
      settings: PreDeleteFcn=|
      | blocks = find_system(gcs, 'SearchDepth', 1, 'Type', 'Block');
      | 
      | for k = 1:length(blocks)
      |     if contains(extractAfter(blocks{k,1}, '/'), 'Source')
      |         set_param(blocks{k}, 'BackgroundColor', '[0.929000, 0.490000, 0.439000]');
      |     end
      | end
  Bus_45 : MATLAB Function  TreatAsAtomicUnit=on  mask{MyInitialization=0, Bus_ID=45, Fault_flag=1}
      mask prompts: Bus_ID "Bus ID"; Fault_flag "Fault flag"
      settings: CopyFcn=|
      | Component_Name = get_param(gcb, 'Name');
      | set_param(gcb, 'Bus_ID', num2str(strtrim(extractAfter(Component_Name, '_'))));
      | 
      | blocks = find_system(gcs, 'SearchDepth', 1, 'Type', 'Block');
      | 
      | for k = 1:length(blocks)
      |     if contains(extractAfter(blocks{k,1}, '/'), 'Source')
      |         set_param(blocks{k}, 'BackgroundColor', '[0.929000, 0.490000, 0.439000]');
      |     end
      | end
      settings: NameChangeFcn=|
      | Component_Name = get_param(gcb, 'Name');
      | old_ID = get_param(gcb, 'Bus_ID');
      | 
      | pattern = '_\d+';
      | match = regexp(Component_Name, pattern, 'match');
      | 
      | if ~isempty(match)
      |     if ~isequal(old_ID, num2str(strtrim(extractAfter(Component_Name, '_'))))
      |         set_param(gcb, 'Bus_ID', num2str(strtrim(extractAfter(Component_Name, '_'))));
      |     end
      | else
      |     newName = [Component_Name '_' old_ID];
      |     set_param(gcb, 'Name', newName);
      | end
      | 
      | if ~isequal(old_ID, get_param(gcb, 'Bus_ID'))
      | 
      |     data = get_param(gcb, 'PortConnectivity');
      |     for i = 1:numel(data)
      |         sourceHandle = data(i,1).SrcBlock;
      |         if ~isempty(sourceHandle) && sourceHandle ~= -1
      |             sourceParams = get_param(sourceHandle, 'DialogParameters');
      |             fn = fieldnames(sourceParams);
      |             if contains(fn{2}, 'Source')
      |                 Bus_ID = get_param(gcb, 'Bus_ID');
      |                 set_param(sourceHandle, 'Source_ID', Bus_ID);
      |             end
      |         end
      |     end
      | 
      |     blocks = find_system(gcs, 'SearchDepth', 1, 'Type', 'Block');
      | 
      |     for k = 1:length(blocks)
      |         if contains(extractAfter(blocks{k,1}, '/'), 'Source')
      |             set_param(blocks{k}, 'BackgroundColor', '[0.929000, 0.490000, 0.439000]');
      |         end
      |     end
      | 
      | end
      settings: PreDeleteFcn=|
      | blocks = find_system(gcs, 'SearchDepth', 1, 'Type', 'Block');
      | 
      | for k = 1:length(blocks)
      |     if contains(extractAfter(blocks{k,1}, '/'), 'Source')
      |         set_param(blocks{k}, 'BackgroundColor', '[0.929000, 0.490000, 0.439000]');
      |     end
      | end
  Bus_46 : MATLAB Function  TreatAsAtomicUnit=on  mask{MyInitialization=0, Bus_ID=46, Fault_flag=1}
      mask prompts: Bus_ID "Bus ID"; Fault_flag "Fault flag"
      settings: CopyFcn=|
      | Component_Name = get_param(gcb, 'Name');
      | set_param(gcb, 'Bus_ID', num2str(strtrim(extractAfter(Component_Name, '_'))));
      | 
      | blocks = find_system(gcs, 'SearchDepth', 1, 'Type', 'Block');
      | 
      | for k = 1:length(blocks)
      |     if contains(extractAfter(blocks{k,1}, '/'), 'Source')
      |         set_param(blocks{k}, 'BackgroundColor', '[0.929000, 0.490000, 0.439000]');
      |     end
      | end
      settings: NameChangeFcn=|
      | Component_Name = get_param(gcb, 'Name');
      | old_ID = get_param(gcb, 'Bus_ID');
      | 
      | pattern = '_\d+';
      | match = regexp(Component_Name, pattern, 'match');
      | 
      | if ~isempty(match)
      |     if ~isequal(old_ID, num2str(strtrim(extractAfter(Component_Name, '_'))))
      |         set_param(gcb, 'Bus_ID', num2str(strtrim(extractAfter(Component_Name, '_'))));
      |     end
      | else
      |     newName = [Component_Name '_' old_ID];
      |     set_param(gcb, 'Name', newName);
      | end
      | 
      | if ~isequal(old_ID, get_param(gcb, 'Bus_ID'))
      | 
      |     data = get_param(gcb, 'PortConnectivity');
      |     for i = 1:numel(data)
      |         sourceHandle = data(i,1).SrcBlock;
      |         if ~isempty(sourceHandle) && sourceHandle ~= -1
      |             sourceParams = get_param(sourceHandle, 'DialogParameters');
      |             fn = fieldnames(sourceParams);
      |             if contains(fn{2}, 'Source')
      |                 Bus_ID = get_param(gcb, 'Bus_ID');
      |                 set_param(sourceHandle, 'Source_ID', Bus_ID);
      |             end
      |         end
      |     end
      | 
      |     blocks = find_system(gcs, 'SearchDepth', 1, 'Type', 'Block');
      | 
      |     for k = 1:length(blocks)
      |         if contains(extractAfter(blocks{k,1}, '/'), 'Source')
      |             set_param(blocks{k}, 'BackgroundColor', '[0.929000, 0.490000, 0.439000]');
      |         end
      |     end
      | 
      | end
      settings: PreDeleteFcn=|
      | blocks = find_system(gcs, 'SearchDepth', 1, 'Type', 'Block');
      | 
      | for k = 1:length(blocks)
      |     if contains(extractAfter(blocks{k,1}, '/'), 'Source')
      |         set_param(blocks{k}, 'BackgroundColor', '[0.929000, 0.490000, 0.439000]');
      |     end
      | end
  Bus_47 : MATLAB Function  TreatAsAtomicUnit=on  mask{MyInitialization=0, Bus_ID=47, Fault_flag=1}
      mask prompts: Bus_ID "Bus ID"; Fault_flag "Fault flag"
      settings: CopyFcn=|
      | Component_Name = get_param(gcb, 'Name');
      | set_param(gcb, 'Bus_ID', num2str(strtrim(extractAfter(Component_Name, '_'))));
      | 
      | blocks = find_system(gcs, 'SearchDepth', 1, 'Type', 'Block');
      | 
      | for k = 1:length(blocks)
      |     if contains(extractAfter(blocks{k,1}, '/'), 'Source')
      |         set_param(blocks{k}, 'BackgroundColor', '[0.929000, 0.490000, 0.439000]');
      |     end
      | end
      settings: NameChangeFcn=|
      | Component_Name = get_param(gcb, 'Name');
      | old_ID = get_param(gcb, 'Bus_ID');
      | 
      | pattern = '_\d+';
      | match = regexp(Component_Name, pattern, 'match');
      | 
      | if ~isempty(match)
      |     if ~isequal(old_ID, num2str(strtrim(extractAfter(Component_Name, '_'))))
      |         set_param(gcb, 'Bus_ID', num2str(strtrim(extractAfter(Component_Name, '_'))));
      |     end
      | else
      |     newName = [Component_Name '_' old_ID];
      |     set_param(gcb, 'Name', newName);
      | end
      | 
      | if ~isequal(old_ID, get_param(gcb, 'Bus_ID'))
      | 
      |     data = get_param(gcb, 'PortConnectivity');
      |     for i = 1:numel(data)
      |         sourceHandle = data(i,1).SrcBlock;
      |         if ~isempty(sourceHandle) && sourceHandle ~= -1
      |             sourceParams = get_param(sourceHandle, 'DialogParameters');
      |             fn = fieldnames(sourceParams);
      |             if contains(fn{2}, 'Source')
      |                 Bus_ID = get_param(gcb, 'Bus_ID');
      |                 set_param(sourceHandle, 'Source_ID', Bus_ID);
      |             end
      |         end
      |     end
      | 
      |     blocks = find_system(gcs, 'SearchDepth', 1, 'Type', 'Block');
      | 
      |     for k = 1:length(blocks)
      |         if contains(extractAfter(blocks{k,1}, '/'), 'Source')
      |             set_param(blocks{k}, 'BackgroundColor', '[0.929000, 0.490000, 0.439000]');
      |         end
      |     end
      | 
      | end
      settings: PreDeleteFcn=|
      | blocks = find_system(gcs, 'SearchDepth', 1, 'Type', 'Block');
      | 
      | for k = 1:length(blocks)
      |     if contains(extractAfter(blocks{k,1}, '/'), 'Source')
      |         set_param(blocks{k}, 'BackgroundColor', '[0.929000, 0.490000, 0.439000]');
      |     end
      | end
  Bus_48 : MATLAB Function  TreatAsAtomicUnit=on  mask{MyInitialization=0, Bus_ID=48, Fault_flag=1}
      mask prompts: Bus_ID "Bus ID"; Fault_flag "Fault flag"
      settings: CopyFcn=|
      | Component_Name = get_param(gcb, 'Name');
      | set_param(gcb, 'Bus_ID', num2str(strtrim(extractAfter(Component_Name, '_'))));
      | 
      | blocks = find_system(gcs, 'SearchDepth', 1, 'Type', 'Block');
      | 
      | for k = 1:length(blocks)
      |     if contains(extractAfter(blocks{k,1}, '/'), 'Source')
      |         set_param(blocks{k}, 'BackgroundColor', '[0.929000, 0.490000, 0.439000]');
      |     end
      | end
      settings: NameChangeFcn=|
      | Component_Name = get_param(gcb, 'Name');
      | old_ID = get_param(gcb, 'Bus_ID');
      | 
      | pattern = '_\d+';
      | match = regexp(Component_Name, pattern, 'match');
      | 
      | if ~isempty(match)
      |     if ~isequal(old_ID, num2str(strtrim(extractAfter(Component_Name, '_'))))
      |         set_param(gcb, 'Bus_ID', num2str(strtrim(extractAfter(Component_Name, '_'))));
      |     end
      | else
      |     newName = [Component_Name '_' old_ID];
      |     set_param(gcb, 'Name', newName);
      | end
      | 
      | if ~isequal(old_ID, get_param(gcb, 'Bus_ID'))
      | 
      |     data = get_param(gcb, 'PortConnectivity');
      |     for i = 1:numel(data)
      |         sourceHandle = data(i,1).SrcBlock;
      |         if ~isempty(sourceHandle) && sourceHandle ~= -1
      |             sourceParams = get_param(sourceHandle, 'DialogParameters');
      |             fn = fieldnames(sourceParams);
      |             if contains(fn{2}, 'Source')
      |                 Bus_ID = get_param(gcb, 'Bus_ID');
      |                 set_param(sourceHandle, 'Source_ID', Bus_ID);
      |             end
      |         end
      |     end
      | 
      |     blocks = find_system(gcs, 'SearchDepth', 1, 'Type', 'Block');
      | 
      |     for k = 1:length(blocks)
      |         if contains(extractAfter(blocks{k,1}, '/'), 'Source')
      |             set_param(blocks{k}, 'BackgroundColor', '[0.929000, 0.490000, 0.439000]');
      |         end
      |     end
      | 
      | end
      settings: PreDeleteFcn=|
      | blocks = find_system(gcs, 'SearchDepth', 1, 'Type', 'Block');
      | 
      | for k = 1:length(blocks)
      |     if contains(extractAfter(blocks{k,1}, '/'), 'Source')
      |         set_param(blocks{k}, 'BackgroundColor', '[0.929000, 0.490000, 0.439000]');
      |     end
      | end
  Bus_49 : MATLAB Function  TreatAsAtomicUnit=on  mask{MyInitialization=0, Bus_ID=49, Fault_flag=1}
      mask prompts: Bus_ID "Bus ID"; Fault_flag "Fault flag"
      settings: CopyFcn=|
      | Component_Name = get_param(gcb, 'Name');
      | set_param(gcb, 'Bus_ID', num2str(strtrim(extractAfter(Component_Name, '_'))));
      | 
      | blocks = find_system(gcs, 'SearchDepth', 1, 'Type', 'Block');
      | 
      | for k = 1:length(blocks)
      |     if contains(extractAfter(blocks{k,1}, '/'), 'Source')
      |         set_param(blocks{k}, 'BackgroundColor', '[0.929000, 0.490000, 0.439000]');
      |     end
      | end
      settings: NameChangeFcn=|
      | Component_Name = get_param(gcb, 'Name');
      | old_ID = get_param(gcb, 'Bus_ID');
      | 
      | pattern = '_\d+';
      | match = regexp(Component_Name, pattern, 'match');
      | 
      | if ~isempty(match)
      |     if ~isequal(old_ID, num2str(strtrim(extractAfter(Component_Name, '_'))))
      |         set_param(gcb, 'Bus_ID', num2str(strtrim(extractAfter(Component_Name, '_'))));
      |     end
      | else
      |     newName = [Component_Name '_' old_ID];
      |     set_param(gcb, 'Name', newName);
      | end
      | 
      | if ~isequal(old_ID, get_param(gcb, 'Bus_ID'))
      | 
      |     data = get_param(gcb, 'PortConnectivity');
      |     for i = 1:numel(data)
      |         sourceHandle = data(i,1).SrcBlock;
      |         if ~isempty(sourceHandle) && sourceHandle ~= -1
      |             sourceParams = get_param(sourceHandle, 'DialogParameters');
      |             fn = fieldnames(sourceParams);
      |             if contains(fn{2}, 'Source')
      |                 Bus_ID = get_param(gcb, 'Bus_ID');
      |                 set_param(sourceHandle, 'Source_ID', Bus_ID);
      |             end
      |         end
      |     end
      | 
      |     blocks = find_system(gcs, 'SearchDepth', 1, 'Type', 'Block');
      | 
      |     for k = 1:length(blocks)
      |         if contains(extractAfter(blocks{k,1}, '/'), 'Source')
      |             set_param(blocks{k}, 'BackgroundColor', '[0.929000, 0.490000, 0.439000]');
      |         end
      |     end
      | 
      | end
      settings: PreDeleteFcn=|
      | blocks = find_system(gcs, 'SearchDepth', 1, 'Type', 'Block');
      | 
      | for k = 1:length(blocks)
      |     if contains(extractAfter(blocks{k,1}, '/'), 'Source')
      |         set_param(blocks{k}, 'BackgroundColor', '[0.929000, 0.490000, 0.439000]');
      |     end
      | end
  Bus_5 : MATLAB Function  TreatAsAtomicUnit=on  mask{MyInitialization=0, Bus_ID=5, Fault_flag=1}
      mask prompts: Bus_ID "Bus ID"; Fault_flag "Fault flag"
      settings: CopyFcn=|
      | Component_Name = get_param(gcb, 'Name');
      | set_param(gcb, 'Bus_ID', num2str(strtrim(extractAfter(Component_Name, '_'))));
      | 
      | blocks = find_system(gcs, 'SearchDepth', 1, 'Type', 'Block');
      | 
      | for k = 1:length(blocks)
      |     if contains(extractAfter(blocks{k,1}, '/'), 'Source')
      |         set_param(blocks{k}, 'BackgroundColor', '[0.929000, 0.490000, 0.439000]');
      |     end
      | end
      settings: NameChangeFcn=|
      | Component_Name = get_param(gcb, 'Name');
      | old_ID = get_param(gcb, 'Bus_ID');
      | 
      | pattern = '_\d+';
      | match = regexp(Component_Name, pattern, 'match');
      | 
      | if ~isempty(match)
      |     if ~isequal(old_ID, num2str(strtrim(extractAfter(Component_Name, '_'))))
      |         set_param(gcb, 'Bus_ID', num2str(strtrim(extractAfter(Component_Name, '_'))));
      |     end
      | else
      |     newName = [Component_Name '_' old_ID];
      |     set_param(gcb, 'Name', newName);
      | end
      | 
      | if ~isequal(old_ID, get_param(gcb, 'Bus_ID'))
      | 
      |     data = get_param(gcb, 'PortConnectivity');
      |     for i = 1:numel(data)
      |         sourceHandle = data(i,1).SrcBlock;
      |         if ~isempty(sourceHandle) && sourceHandle ~= -1
      |             sourceParams = get_param(sourceHandle, 'DialogParameters');
      |             fn = fieldnames(sourceParams);
      |             if contains(fn{2}, 'Source')
      |                 Bus_ID = get_param(gcb, 'Bus_ID');
      |                 set_param(sourceHandle, 'Source_ID', Bus_ID);
      |             end
      |         end
      |     end
      | 
      |     blocks = find_system(gcs, 'SearchDepth', 1, 'Type', 'Block');
      | 
      |     for k = 1:length(blocks)
      |         if contains(extractAfter(blocks{k,1}, '/'), 'Source')
      |             set_param(blocks{k}, 'BackgroundColor', '[0.929000, 0.490000, 0.439000]');
      |         end
      |     end
      | 
      | end
      settings: PreDeleteFcn=|
      | blocks = find_system(gcs, 'SearchDepth', 1, 'Type', 'Block');
      | 
      | for k = 1:length(blocks)
      |     if contains(extractAfter(blocks{k,1}, '/'), 'Source')
      |         set_param(blocks{k}, 'BackgroundColor', '[0.929000, 0.490000, 0.439000]');
      |     end
      | end
  Bus_50 : MATLAB Function  TreatAsAtomicUnit=on  mask{MyInitialization=0, Bus_ID=50, Fault_flag=0}
      mask prompts: Bus_ID "Bus ID"; Fault_flag "Fault flag"
      settings: CopyFcn=|
      | Component_Name = get_param(gcb, 'Name');
      | set_param(gcb, 'Bus_ID', num2str(strtrim(extractAfter(Component_Name, '_'))));
      | 
      | blocks = find_system(gcs, 'SearchDepth', 1, 'Type', 'Block');
      | 
      | for k = 1:length(blocks)
      |     if contains(extractAfter(blocks{k,1}, '/'), 'Source')
      |         set_param(blocks{k}, 'BackgroundColor', '[0.929000, 0.490000, 0.439000]');
      |     end
      | end
      settings: NameChangeFcn=|
      | Component_Name = get_param(gcb, 'Name');
      | old_ID = get_param(gcb, 'Bus_ID');
      | 
      | pattern = '_\d+';
      | match = regexp(Component_Name, pattern, 'match');
      | 
      | if ~isempty(match)
      |     if ~isequal(old_ID, num2str(strtrim(extractAfter(Component_Name, '_'))))
      |         set_param(gcb, 'Bus_ID', num2str(strtrim(extractAfter(Component_Name, '_'))));
      |     end
      | else
      |     newName = [Component_Name '_' old_ID];
      |     set_param(gcb, 'Name', newName);
      | end
      | 
      | if ~isequal(old_ID, get_param(gcb, 'Bus_ID'))
      | 
      |     data = get_param(gcb, 'PortConnectivity');
      |     for i = 1:numel(data)
      |         sourceHandle = data(i,1).SrcBlock;
      |         if ~isempty(sourceHandle) && sourceHandle ~= -1
      |             sourceParams = get_param(sourceHandle, 'DialogParameters');
      |             fn = fieldnames(sourceParams);
      |             if contains(fn{2}, 'Source')
      |                 Bus_ID = get_param(gcb, 'Bus_ID');
      |                 set_param(sourceHandle, 'Source_ID', Bus_ID);
      |             end
      |         end
      |     end
      | 
      |     blocks = find_system(gcs, 'SearchDepth', 1, 'Type', 'Block');
      | 
      |     for k = 1:length(blocks)
      |         if contains(extractAfter(blocks{k,1}, '/'), 'Source')
      |             set_param(blocks{k}, 'BackgroundColor', '[0.929000, 0.490000, 0.439000]');
      |         end
      |     end
      | 
      | end
      settings: PreDeleteFcn=|
      | blocks = find_system(gcs, 'SearchDepth', 1, 'Type', 'Block');
      | 
      | for k = 1:length(blocks)
      |     if contains(extractAfter(blocks{k,1}, '/'), 'Source')
      |         set_param(blocks{k}, 'BackgroundColor', '[0.929000, 0.490000, 0.439000]');
      |     end
      | end
  Bus_51 : MATLAB Function  TreatAsAtomicUnit=on  mask{MyInitialization=0, Bus_ID=51, Fault_flag=1}
      mask prompts: Bus_ID "Bus ID"; Fault_flag "Fault flag"
      settings: CopyFcn=|
      | Component_Name = get_param(gcb, 'Name');
      | set_param(gcb, 'Bus_ID', num2str(strtrim(extractAfter(Component_Name, '_'))));
      | 
      | blocks = find_system(gcs, 'SearchDepth', 1, 'Type', 'Block');
      | 
      | for k = 1:length(blocks)
      |     if contains(extractAfter(blocks{k,1}, '/'), 'Source')
      |         set_param(blocks{k}, 'BackgroundColor', '[0.929000, 0.490000, 0.439000]');
      |     end
      | end
      settings: NameChangeFcn=|
      | Component_Name = get_param(gcb, 'Name');
      | old_ID = get_param(gcb, 'Bus_ID');
      | 
      | pattern = '_\d+';
      | match = regexp(Component_Name, pattern, 'match');
      | 
      | if ~isempty(match)
      |     if ~isequal(old_ID, num2str(strtrim(extractAfter(Component_Name, '_'))))
      |         set_param(gcb, 'Bus_ID', num2str(strtrim(extractAfter(Component_Name, '_'))));
      |     end
      | else
      |     newName = [Component_Name '_' old_ID];
      |     set_param(gcb, 'Name', newName);
      | end
      | 
      | if ~isequal(old_ID, get_param(gcb, 'Bus_ID'))
      | 
      |     data = get_param(gcb, 'PortConnectivity');
      |     for i = 1:numel(data)
      |         sourceHandle = data(i,1).SrcBlock;
      |         if ~isempty(sourceHandle) && sourceHandle ~= -1
      |             sourceParams = get_param(sourceHandle, 'DialogParameters');
      |             fn = fieldnames(sourceParams);
      |             if contains(fn{2}, 'Source')
      |                 Bus_ID = get_param(gcb, 'Bus_ID');
      |                 set_param(sourceHandle, 'Source_ID', Bus_ID);
      |             end
      |         end
      |     end
      | 
      |     blocks = find_system(gcs, 'SearchDepth', 1, 'Type', 'Block');
      | 
      |     for k = 1:length(blocks)
      |         if contains(extractAfter(blocks{k,1}, '/'), 'Source')
      |             set_param(blocks{k}, 'BackgroundColor', '[0.929000, 0.490000, 0.439000]');
      |         end
      |     end
      | 
      | end
      settings: PreDeleteFcn=|
      | blocks = find_system(gcs, 'SearchDepth', 1, 'Type', 'Block');
      | 
      | for k = 1:length(blocks)
      |     if contains(extractAfter(blocks{k,1}, '/'), 'Source')
      |         set_param(blocks{k}, 'BackgroundColor', '[0.929000, 0.490000, 0.439000]');
      |     end
      | end
  Bus_52 : MATLAB Function  TreatAsAtomicUnit=on  mask{MyInitialization=0, Bus_ID=52, Fault_flag=0}
      mask prompts: Bus_ID "Bus ID"; Fault_flag "Fault flag"
      settings: CopyFcn=|
      | Component_Name = get_param(gcb, 'Name');
      | set_param(gcb, 'Bus_ID', num2str(strtrim(extractAfter(Component_Name, '_'))));
      | 
      | blocks = find_system(gcs, 'SearchDepth', 1, 'Type', 'Block');
      | 
      | for k = 1:length(blocks)
      |     if contains(extractAfter(blocks{k,1}, '/'), 'Source')
      |         set_param(blocks{k}, 'BackgroundColor', '[0.929000, 0.490000, 0.439000]');
      |     end
      | end
      settings: NameChangeFcn=|
      | Component_Name = get_param(gcb, 'Name');
      | old_ID = get_param(gcb, 'Bus_ID');
      | 
      | pattern = '_\d+';
      | match = regexp(Component_Name, pattern, 'match');
      | 
      | if ~isempty(match)
      |     if ~isequal(old_ID, num2str(strtrim(extractAfter(Component_Name, '_'))))
      |         set_param(gcb, 'Bus_ID', num2str(strtrim(extractAfter(Component_Name, '_'))));
      |     end
      | else
      |     newName = [Component_Name '_' old_ID];
      |     set_param(gcb, 'Name', newName);
      | end
      | 
      | if ~isequal(old_ID, get_param(gcb, 'Bus_ID'))
      | 
      |     data = get_param(gcb, 'PortConnectivity');
      |     for i = 1:numel(data)
      |         sourceHandle = data(i,1).SrcBlock;
      |         if ~isempty(sourceHandle) && sourceHandle ~= -1
      |             sourceParams = get_param(sourceHandle, 'DialogParameters');
      |             fn = fieldnames(sourceParams);
      |             if contains(fn{2}, 'Source')
      |                 Bus_ID = get_param(gcb, 'Bus_ID');
      |                 set_param(sourceHandle, 'Source_ID', Bus_ID);
      |             end
      |         end
      |     end
      | 
      |     blocks = find_system(gcs, 'SearchDepth', 1, 'Type', 'Block');
      | 
      |     for k = 1:length(blocks)
      |         if contains(extractAfter(blocks{k,1}, '/'), 'Source')
      |             set_param(blocks{k}, 'BackgroundColor', '[0.929000, 0.490000, 0.439000]');
      |         end
      |     end
      | 
      | end
      settings: PreDeleteFcn=|
      | blocks = find_system(gcs, 'SearchDepth', 1, 'Type', 'Block');
      | 
      | for k = 1:length(blocks)
      |     if contains(extractAfter(blocks{k,1}, '/'), 'Source')
      |         set_param(blocks{k}, 'BackgroundColor', '[0.929000, 0.490000, 0.439000]');
      |     end
      | end
  Bus_53 : MATLAB Function  TreatAsAtomicUnit=on  mask{MyInitialization=0, Bus_ID=53, Fault_flag=0}
      mask prompts: Bus_ID "Bus ID"; Fault_flag "Fault flag"
      settings: CopyFcn=|
      | Component_Name = get_param(gcb, 'Name');
      | set_param(gcb, 'Bus_ID', num2str(strtrim(extractAfter(Component_Name, '_'))));
      | 
      | blocks = find_system(gcs, 'SearchDepth', 1, 'Type', 'Block');
      | 
      | for k = 1:length(blocks)
      |     if contains(extractAfter(blocks{k,1}, '/'), 'Source')
      |         set_param(blocks{k}, 'BackgroundColor', '[0.929000, 0.490000, 0.439000]');
      |     end
      | end
      settings: NameChangeFcn=|
      | Component_Name = get_param(gcb, 'Name');
      | old_ID = get_param(gcb, 'Bus_ID');
      | 
      | pattern = '_\d+';
      | match = regexp(Component_Name, pattern, 'match');
      | 
      | if ~isempty(match)
      |     if ~isequal(old_ID, num2str(strtrim(extractAfter(Component_Name, '_'))))
      |         set_param(gcb, 'Bus_ID', num2str(strtrim(extractAfter(Component_Name, '_'))));
      |     end
      | else
      |     newName = [Component_Name '_' old_ID];
      |     set_param(gcb, 'Name', newName);
      | end
      | 
      | if ~isequal(old_ID, get_param(gcb, 'Bus_ID'))
      | 
      |     data = get_param(gcb, 'PortConnectivity');
      |     for i = 1:numel(data)
      |         sourceHandle = data(i,1).SrcBlock;
      |         if ~isempty(sourceHandle) && sourceHandle ~= -1
      |             sourceParams = get_param(sourceHandle, 'DialogParameters');
      |             fn = fieldnames(sourceParams);
      |             if contains(fn{2}, 'Source')
      |                 Bus_ID = get_param(gcb, 'Bus_ID');
      |                 set_param(sourceHandle, 'Source_ID', Bus_ID);
      |             end
      |         end
      |     end
      | 
      |     blocks = find_system(gcs, 'SearchDepth', 1, 'Type', 'Block');
      | 
      |     for k = 1:length(blocks)
      |         if contains(extractAfter(blocks{k,1}, '/'), 'Source')
      |             set_param(blocks{k}, 'BackgroundColor', '[0.929000, 0.490000, 0.439000]');
      |         end
      |     end
      | 
      | end
      settings: PreDeleteFcn=|
      | blocks = find_system(gcs, 'SearchDepth', 1, 'Type', 'Block');
      | 
      | for k = 1:length(blocks)
      |     if contains(extractAfter(blocks{k,1}, '/'), 'Source')
      |         set_param(blocks{k}, 'BackgroundColor', '[0.929000, 0.490000, 0.439000]');
      |     end
      | end
  Bus_54 : MATLAB Function  TreatAsAtomicUnit=on  mask{MyInitialization=0, Bus_ID=54, Fault_flag=1}
      mask prompts: Bus_ID "Bus ID"; Fault_flag "Fault flag"
      settings: CopyFcn=|
      | Component_Name = get_param(gcb, 'Name');
      | set_param(gcb, 'Bus_ID', num2str(strtrim(extractAfter(Component_Name, '_'))));
      | 
      | blocks = find_system(gcs, 'SearchDepth', 1, 'Type', 'Block');
      | 
      | for k = 1:length(blocks)
      |     if contains(extractAfter(blocks{k,1}, '/'), 'Source')
      |         set_param(blocks{k}, 'BackgroundColor', '[0.929000, 0.490000, 0.439000]');
      |     end
      | end
      settings: NameChangeFcn=|
      | Component_Name = get_param(gcb, 'Name');
      | old_ID = get_param(gcb, 'Bus_ID');
      | 
      | pattern = '_\d+';
      | match = regexp(Component_Name, pattern, 'match');
      | 
      | if ~isempty(match)
      |     if ~isequal(old_ID, num2str(strtrim(extractAfter(Component_Name, '_'))))
      |         set_param(gcb, 'Bus_ID', num2str(strtrim(extractAfter(Component_Name, '_'))));
      |     end
      | else
      |     newName = [Component_Name '_' old_ID];
      |     set_param(gcb, 'Name', newName);
      | end
      | 
      | if ~isequal(old_ID, get_param(gcb, 'Bus_ID'))
      | 
      |     data = get_param(gcb, 'PortConnectivity');
      |     for i = 1:numel(data)
      |         sourceHandle = data(i,1).SrcBlock;
      |         if ~isempty(sourceHandle) && sourceHandle ~= -1
      |             sourceParams = get_param(sourceHandle, 'DialogParameters');
      |             fn = fieldnames(sourceParams);
      |             if contains(fn{2}, 'Source')
      |                 Bus_ID = get_param(gcb, 'Bus_ID');
      |                 set_param(sourceHandle, 'Source_ID', Bus_ID);
      |             end
      |         end
      |     end
      | 
      |     blocks = find_system(gcs, 'SearchDepth', 1, 'Type', 'Block');
      | 
      |     for k = 1:length(blocks)
      |         if contains(extractAfter(blocks{k,1}, '/'), 'Source')
      |             set_param(blocks{k}, 'BackgroundColor', '[0.929000, 0.490000, 0.439000]');
      |         end
      |     end
      | 
      | end
      settings: PreDeleteFcn=|
      | blocks = find_system(gcs, 'SearchDepth', 1, 'Type', 'Block');
      | 
      | for k = 1:length(blocks)
      |     if contains(extractAfter(blocks{k,1}, '/'), 'Source')
      |         set_param(blocks{k}, 'BackgroundColor', '[0.929000, 0.490000, 0.439000]');
      |     end
      | end
  Bus_55 : MATLAB Function  TreatAsAtomicUnit=on  mask{MyInitialization=0, Bus_ID=55, Fault_flag=1}
      mask prompts: Bus_ID "Bus ID"; Fault_flag "Fault flag"
      settings: CopyFcn=|
      | Component_Name = get_param(gcb, 'Name');
      | set_param(gcb, 'Bus_ID', num2str(strtrim(extractAfter(Component_Name, '_'))));
      | 
      | blocks = find_system(gcs, 'SearchDepth', 1, 'Type', 'Block');
      | 
      | for k = 1:length(blocks)
      |     if contains(extractAfter(blocks{k,1}, '/'), 'Source')
      |         set_param(blocks{k}, 'BackgroundColor', '[0.929000, 0.490000, 0.439000]');
      |     end
      | end
      settings: NameChangeFcn=|
      | Component_Name = get_param(gcb, 'Name');
      | old_ID = get_param(gcb, 'Bus_ID');
      | 
      | pattern = '_\d+';
      | match = regexp(Component_Name, pattern, 'match');
      | 
      | if ~isempty(match)
      |     if ~isequal(old_ID, num2str(strtrim(extractAfter(Component_Name, '_'))))
      |         set_param(gcb, 'Bus_ID', num2str(strtrim(extractAfter(Component_Name, '_'))));
      |     end
      | else
      |     newName = [Component_Name '_' old_ID];
      |     set_param(gcb, 'Name', newName);
      | end
      | 
      | if ~isequal(old_ID, get_param(gcb, 'Bus_ID'))
      | 
      |     data = get_param(gcb, 'PortConnectivity');
      |     for i = 1:numel(data)
      |         sourceHandle = data(i,1).SrcBlock;
      |         if ~isempty(sourceHandle) && sourceHandle ~= -1
      |             sourceParams = get_param(sourceHandle, 'DialogParameters');
      |             fn = fieldnames(sourceParams);
      |             if contains(fn{2}, 'Source')
      |                 Bus_ID = get_param(gcb, 'Bus_ID');
      |                 set_param(sourceHandle, 'Source_ID', Bus_ID);
      |             end
      |         end
      |     end
      | 
      |     blocks = find_system(gcs, 'SearchDepth', 1, 'Type', 'Block');
      | 
      |     for k = 1:length(blocks)
      |         if contains(extractAfter(blocks{k,1}, '/'), 'Source')
      |             set_param(blocks{k}, 'BackgroundColor', '[0.929000, 0.490000, 0.439000]');
      |         end
      |     end
      | 
      | end
      settings: PreDeleteFcn=|
      | blocks = find_system(gcs, 'SearchDepth', 1, 'Type', 'Block');
      | 
      | for k = 1:length(blocks)
      |     if contains(extractAfter(blocks{k,1}, '/'), 'Source')
      |         set_param(blocks{k}, 'BackgroundColor', '[0.929000, 0.490000, 0.439000]');
      |     end
      | end
  Bus_56 : MATLAB Function  TreatAsAtomicUnit=on  mask{MyInitialization=0, Bus_ID=56, Fault_flag=1}
      mask prompts: Bus_ID "Bus ID"; Fault_flag "Fault flag"
      settings: CopyFcn=|
      | Component_Name = get_param(gcb, 'Name');
      | set_param(gcb, 'Bus_ID', num2str(strtrim(extractAfter(Component_Name, '_'))));
      | 
      | blocks = find_system(gcs, 'SearchDepth', 1, 'Type', 'Block');
      | 
      | for k = 1:length(blocks)
      |     if contains(extractAfter(blocks{k,1}, '/'), 'Source')
      |         set_param(blocks{k}, 'BackgroundColor', '[0.929000, 0.490000, 0.439000]');
      |     end
      | end
      settings: NameChangeFcn=|
      | Component_Name = get_param(gcb, 'Name');
      | old_ID = get_param(gcb, 'Bus_ID');
      | 
      | pattern = '_\d+';
      | match = regexp(Component_Name, pattern, 'match');
      | 
      | if ~isempty(match)
      |     if ~isequal(old_ID, num2str(strtrim(extractAfter(Component_Name, '_'))))
      |         set_param(gcb, 'Bus_ID', num2str(strtrim(extractAfter(Component_Name, '_'))));
      |     end
      | else
      |     newName = [Component_Name '_' old_ID];
      |     set_param(gcb, 'Name', newName);
      | end
      | 
      | if ~isequal(old_ID, get_param(gcb, 'Bus_ID'))
      | 
      |     data = get_param(gcb, 'PortConnectivity');
      |     for i = 1:numel(data)
      |         sourceHandle = data(i,1).SrcBlock;
      |         if ~isempty(sourceHandle) && sourceHandle ~= -1
      |             sourceParams = get_param(sourceHandle, 'DialogParameters');
      |             fn = fieldnames(sourceParams);
      |             if contains(fn{2}, 'Source')
      |                 Bus_ID = get_param(gcb, 'Bus_ID');
      |                 set_param(sourceHandle, 'Source_ID', Bus_ID);
      |             end
      |         end
      |     end
      | 
      |     blocks = find_system(gcs, 'SearchDepth', 1, 'Type', 'Block');
      | 
      |     for k = 1:length(blocks)
      |         if contains(extractAfter(blocks{k,1}, '/'), 'Source')
      |             set_param(blocks{k}, 'BackgroundColor', '[0.929000, 0.490000, 0.439000]');
      |         end
      |     end
      | 
      | end
      settings: PreDeleteFcn=|
      | blocks = find_system(gcs, 'SearchDepth', 1, 'Type', 'Block');
      | 
      | for k = 1:length(blocks)
      |     if contains(extractAfter(blocks{k,1}, '/'), 'Source')
      |         set_param(blocks{k}, 'BackgroundColor', '[0.929000, 0.490000, 0.439000]');
      |     end
      | end
  Bus_57 : MATLAB Function  TreatAsAtomicUnit=on  mask{MyInitialization=0, Bus_ID=57, Fault_flag=1}
      mask prompts: Bus_ID "Bus ID"; Fault_flag "Fault flag"
      settings: CopyFcn=|
      | Component_Name = get_param(gcb, 'Name');
      | set_param(gcb, 'Bus_ID', num2str(strtrim(extractAfter(Component_Name, '_'))));
      | 
      | blocks = find_system(gcs, 'SearchDepth', 1, 'Type', 'Block');
      | 
      | for k = 1:length(blocks)
      |     if contains(extractAfter(blocks{k,1}, '/'), 'Source')
      |         set_param(blocks{k}, 'BackgroundColor', '[0.929000, 0.490000, 0.439000]');
      |     end
      | end
      settings: NameChangeFcn=|
      | Component_Name = get_param(gcb, 'Name');
      | old_ID = get_param(gcb, 'Bus_ID');
      | 
      | pattern = '_\d+';
      | match = regexp(Component_Name, pattern, 'match');
      | 
      | if ~isempty(match)
      |     if ~isequal(old_ID, num2str(strtrim(extractAfter(Component_Name, '_'))))
      |         set_param(gcb, 'Bus_ID', num2str(strtrim(extractAfter(Component_Name, '_'))));
      |     end
      | else
      |     newName = [Component_Name '_' old_ID];
      |     set_param(gcb, 'Name', newName);
      | end
      | 
      | if ~isequal(old_ID, get_param(gcb, 'Bus_ID'))
      | 
      |     data = get_param(gcb, 'PortConnectivity');
      |     for i = 1:numel(data)
      |         sourceHandle = data(i,1).SrcBlock;
      |         if ~isempty(sourceHandle) && sourceHandle ~= -1
      |             sourceParams = get_param(sourceHandle, 'DialogParameters');
      |             fn = fieldnames(sourceParams);
      |             if contains(fn{2}, 'Source')
      |                 Bus_ID = get_param(gcb, 'Bus_ID');
      |                 set_param(sourceHandle, 'Source_ID', Bus_ID);
      |             end
      |         end
      |     end
      | 
      |     blocks = find_system(gcs, 'SearchDepth', 1, 'Type', 'Block');
      | 
      |     for k = 1:length(blocks)
      |         if contains(extractAfter(blocks{k,1}, '/'), 'Source')
      |             set_param(blocks{k}, 'BackgroundColor', '[0.929000, 0.490000, 0.439000]');
      |         end
      |     end
      | 
      | end
      settings: PreDeleteFcn=|
      | blocks = find_system(gcs, 'SearchDepth', 1, 'Type', 'Block');
      | 
      | for k = 1:length(blocks)
      |     if contains(extractAfter(blocks{k,1}, '/'), 'Source')
      |         set_param(blocks{k}, 'BackgroundColor', '[0.929000, 0.490000, 0.439000]');
      |     end
      | end
  Bus_58 : MATLAB Function  TreatAsAtomicUnit=on  mask{MyInitialization=0, Bus_ID=58, Fault_flag=1}
      mask prompts: Bus_ID "Bus ID"; Fault_flag "Fault flag"
      settings: CopyFcn=|
      | Component_Name = get_param(gcb, 'Name');
      | set_param(gcb, 'Bus_ID', num2str(strtrim(extractAfter(Component_Name, '_'))));
      | 
      | blocks = find_system(gcs, 'SearchDepth', 1, 'Type', 'Block');
      | 
      | for k = 1:length(blocks)
      |     if contains(extractAfter(blocks{k,1}, '/'), 'Source')
      |         set_param(blocks{k}, 'BackgroundColor', '[0.929000, 0.490000, 0.439000]');
      |     end
      | end
      settings: NameChangeFcn=|
      | Component_Name = get_param(gcb, 'Name');
      | old_ID = get_param(gcb, 'Bus_ID');
      | 
      | pattern = '_\d+';
      | match = regexp(Component_Name, pattern, 'match');
      | 
      | if ~isempty(match)
      |     if ~isequal(old_ID, num2str(strtrim(extractAfter(Component_Name, '_'))))
      |         set_param(gcb, 'Bus_ID', num2str(strtrim(extractAfter(Component_Name, '_'))));
      |     end
      | else
      |     newName = [Component_Name '_' old_ID];
      |     set_param(gcb, 'Name', newName);
      | end
      | 
      | if ~isequal(old_ID, get_param(gcb, 'Bus_ID'))
      | 
      |     data = get_param(gcb, 'PortConnectivity');
      |     for i = 1:numel(data)
      |         sourceHandle = data(i,1).SrcBlock;
      |         if ~isempty(sourceHandle) && sourceHandle ~= -1
      |             sourceParams = get_param(sourceHandle, 'DialogParameters');
      |             fn = fieldnames(sourceParams);
      |             if contains(fn{2}, 'Source')
      |                 Bus_ID = get_param(gcb, 'Bus_ID');
      |                 set_param(sourceHandle, 'Source_ID', Bus_ID);
      |             end
      |         end
      |     end
      | 
      |     blocks = find_system(gcs, 'SearchDepth', 1, 'Type', 'Block');
      | 
      |     for k = 1:length(blocks)
      |         if contains(extractAfter(blocks{k,1}, '/'), 'Source')
      |             set_param(blocks{k}, 'BackgroundColor', '[0.929000, 0.490000, 0.439000]');
      |         end
      |     end
      | 
      | end
      settings: PreDeleteFcn=|
      | blocks = find_system(gcs, 'SearchDepth', 1, 'Type', 'Block');
      | 
      | for k = 1:length(blocks)
      |     if contains(extractAfter(blocks{k,1}, '/'), 'Source')
      |         set_param(blocks{k}, 'BackgroundColor', '[0.929000, 0.490000, 0.439000]');
      |     end
      | end
  Bus_59 : MATLAB Function  TreatAsAtomicUnit=on  mask{MyInitialization=0, Bus_ID=59, Fault_flag=1}
      mask prompts: Bus_ID "Bus ID"; Fault_flag "Fault flag"
      settings: CopyFcn=|
      | Component_Name = get_param(gcb, 'Name');
      | set_param(gcb, 'Bus_ID', num2str(strtrim(extractAfter(Component_Name, '_'))));
      | 
      | blocks = find_system(gcs, 'SearchDepth', 1, 'Type', 'Block');
      | 
      | for k = 1:length(blocks)
      |     if contains(extractAfter(blocks{k,1}, '/'), 'Source')
      |         set_param(blocks{k}, 'BackgroundColor', '[0.929000, 0.490000, 0.439000]');
      |     end
      | end
      settings: NameChangeFcn=|
      | Component_Name = get_param(gcb, 'Name');
      | old_ID = get_param(gcb, 'Bus_ID');
      | 
      | pattern = '_\d+';
      | match = regexp(Component_Name, pattern, 'match');
      | 
      | if ~isempty(match)
      |     if ~isequal(old_ID, num2str(strtrim(extractAfter(Component_Name, '_'))))
      |         set_param(gcb, 'Bus_ID', num2str(strtrim(extractAfter(Component_Name, '_'))));
      |     end
      | else
      |     newName = [Component_Name '_' old_ID];
      |     set_param(gcb, 'Name', newName);
      | end
      | 
      | if ~isequal(old_ID, get_param(gcb, 'Bus_ID'))
      | 
      |     data = get_param(gcb, 'PortConnectivity');
      |     for i = 1:numel(data)
      |         sourceHandle = data(i,1).SrcBlock;
      |         if ~isempty(sourceHandle) && sourceHandle ~= -1
      |             sourceParams = get_param(sourceHandle, 'DialogParameters');
      |             fn = fieldnames(sourceParams);
      |             if contains(fn{2}, 'Source')
      |                 Bus_ID = get_param(gcb, 'Bus_ID');
      |                 set_param(sourceHandle, 'Source_ID', Bus_ID);
      |             end
      |         end
      |     end
      | 
      |     blocks = find_system(gcs, 'SearchDepth', 1, 'Type', 'Block');
      | 
      |     for k = 1:length(blocks)
      |         if contains(extractAfter(blocks{k,1}, '/'), 'Source')
      |             set_param(blocks{k}, 'BackgroundColor', '[0.929000, 0.490000, 0.439000]');
      |         end
      |     end
      | 
      | end
      settings: PreDeleteFcn=|
      | blocks = find_system(gcs, 'SearchDepth', 1, 'Type', 'Block');
      | 
      | for k = 1:length(blocks)
      |     if contains(extractAfter(blocks{k,1}, '/'), 'Source')
      |         set_param(blocks{k}, 'BackgroundColor', '[0.929000, 0.490000, 0.439000]');
      |     end
      | end
  Bus_6 : MATLAB Function  TreatAsAtomicUnit=on  mask{MyInitialization=0, Bus_ID=6, Fault_flag=1}
      mask prompts: Bus_ID "Bus ID"; Fault_flag "Fault flag"
      settings: CopyFcn=|
      | Component_Name = get_param(gcb, 'Name');
      | set_param(gcb, 'Bus_ID', num2str(strtrim(extractAfter(Component_Name, '_'))));
      | 
      | blocks = find_system(gcs, 'SearchDepth', 1, 'Type', 'Block');
      | 
      | for k = 1:length(blocks)
